simulink model "IEEE68"  (R2024b)
settings: Solver=FixedStepAuto  StartTime=0  StopTime=20  FixedStep=Ts  RelTol=1e-3
undefined symbols (not defined in the file): ApparatusDiscreDamping, ApparatusPara, ApparatusPowerFlow, ApparatusType, Fbase, OtherInputs, Sbase, Ts, Vbase, Wbase, x_e, Ybase, Zbase
libraries: spsGroundLib x101, SimplusGT x98, spsThreePhaseSeriesRLCBranchLib x83, spsThreePhaseParallelRLCBranchLib x71, spsThreePhaseTransformerTwoWindingsLib x16, spsThreePhaseBreakerLib x3, sps_lib x1
settings Model: Creator=tim  LastModifiedBy=tim

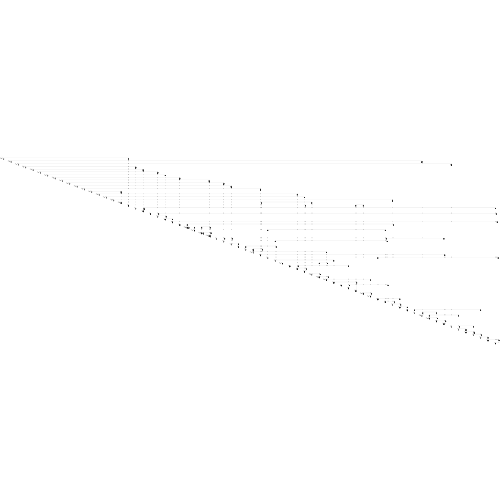
[thumbnail: Simulink's stored preview of the top-level diagram]
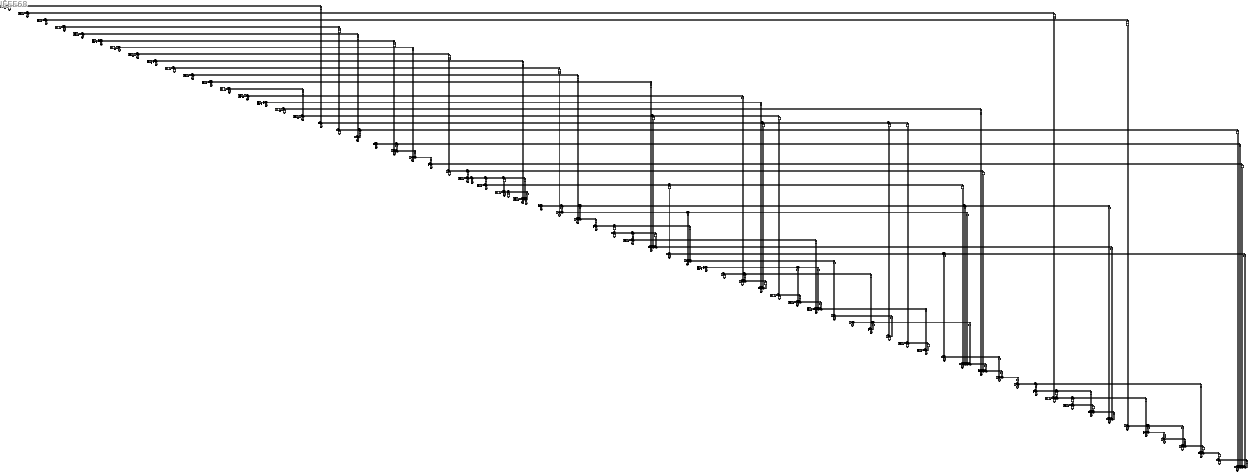
== system IEEE68 ==
  B-GND{1..7,9,11,13,15,17,19,21,23,25,27,29,31,33,36,40,43..44,47,49,51,53,56,60,63,65..66,71,74,76,79,82,84,86,89,91,94,97,99..100,102,104,106,108,111..113,115..116,118,120,122,124,127,130,133,135,137..138,141,143,145,147,149,151} (71 alike) : spsGroundLib/Ground  LConnTagsString=a
  Branch1-1 : spsThreePhaseParallelRLCBranchLib/Three-Phase Parallel RLC Branch  LConnTagsString=A|B|C  RConnTagsString=A|B|C  BranchType=C  Resistance=(Inf)*Zbase  Inductance=(Inf)*Zbase/Wbase  Capacitance=(5e-08)*Ybase/Wbase  Measurements=None
  Branch1-18 : spsThreePhaseSeriesRLCBranchLib/Three-Phase Series RLC Branch  LConnTagsString=A|B|C  RConnTagsString=A|B|C  BranchType=RL  Resistance=(1e-07)*Zbase  Inductance=(0.003)*Zbase/Wbase  Capacitance=1e-6  Measurements=None
  Branch10-10 : spsThreePhaseParallelRLCBranchLib/Three-Phase Parallel RLC Branch  LConnTagsString=A|B|C  RConnTagsString=A|B|C  BranchType=C  Resistance=(Inf)*Zbase  Inductance=(Inf)*Zbase/Wbase  Capacitance=(5e-08)*Ybase/Wbase  Measurements=None
  Branch10-31 : spsThreePhaseSeriesRLCBranchLib/Three-Phase Series RLC Branch  LConnTagsString=A|B|C  RConnTagsString=A|B|C  BranchType=RL  Resistance=(1e-07)*Zbase  Inductance=(0.026)*Zbase/Wbase  Capacitance=1e-6  Measurements=None
  Branch11-11 : spsThreePhaseParallelRLCBranchLib/Three-Phase Parallel RLC Branch  LConnTagsString=A|B|C  RConnTagsString=A|B|C  BranchType=C  Resistance=(Inf)*Zbase  Inductance=(Inf)*Zbase/Wbase  Capacitance=(5e-08)*Ybase/Wbase  Measurements=None
  Branch11-32 : spsThreePhaseSeriesRLCBranchLib/Three-Phase Series RLC Branch  LConnTagsString=A|B|C  RConnTagsString=A|B|C  BranchType=RL  Resistance=(1e-07)*Zbase  Inductance=(0.013)*Zbase/Wbase  Capacitance=1e-6  Measurements=None
  Branch12-12 : spsThreePhaseParallelRLCBranchLib/Three-Phase Parallel RLC Branch  LConnTagsString=A|B|C  RConnTagsString=A|B|C  BranchType=C  Resistance=(Inf)*Zbase  Inductance=(Inf)*Zbase/Wbase  Capacitance=(5e-08)*Ybase/Wbase  Measurements=None
  Branch12-36 : spsThreePhaseSeriesRLCBranchLib/Three-Phase Series RLC Branch  LConnTagsString=A|B|C  RConnTagsString=A|B|C  BranchType=RL  Resistance=(1e-07)*Zbase  Inductance=(0.0075)*Zbase/Wbase  Capacitance=1e-6  Measurements=None
  Branch13-13 : spsThreePhaseParallelRLCBranchLib/Three-Phase Parallel RLC Branch  LConnTagsString=A|B|C  RConnTagsString=A|B|C  BranchType=C  Resistance=(Inf)*Zbase  Inductance=(Inf)*Zbase/Wbase  Capacitance=(5e-08)*Ybase/Wbase  Measurements=None
  Branch13-17 : spsThreePhaseSeriesRLCBranchLib/Three-Phase Series RLC Branch  LConnTagsString=A|B|C  RConnTagsString=A|B|C  BranchType=RL  Resistance=(1e-07)*Zbase  Inductance=(0.0033)*Zbase/Wbase  Capacitance=1e-6  Measurements=None
  Branch14-14 : spsThreePhaseParallelRLCBranchLib/Three-Phase Parallel RLC Branch  LConnTagsString=A|B|C  RConnTagsString=A|B|C  BranchType=C  Resistance=(Inf)*Zbase  Inductance=(Inf)*Zbase/Wbase  Capacitance=(5e-08)*Ybase/Wbase  Measurements=None
  Branch14-41 : spsThreePhaseSeriesRLCBranchLib/Three-Phase Series RLC Branch  LConnTagsString=A|B|C  RConnTagsString=A|B|C  BranchType=RL  Resistance=(1e-07)*Zbase  Inductance=(0.0015)*Zbase/Wbase  Capacitance=1e-6  Measurements=None
  Branch15-15 : spsThreePhaseParallelRLCBranchLib/Three-Phase Parallel RLC Branch  LConnTagsString=A|B|C  RConnTagsString=A|B|C  BranchType=C  Resistance=(Inf)*Zbase  Inductance=(Inf)*Zbase/Wbase  Capacitance=(5e-08)*Ybase/Wbase  Measurements=None
  Branch15-42 : spsThreePhaseSeriesRLCBranchLib/Three-Phase Series RLC Branch  LConnTagsString=A|B|C  RConnTagsString=A|B|C  BranchType=RL  Resistance=(1e-07)*Zbase  Inductance=(0.0015)*Zbase/Wbase  Capacitance=1e-6  Measurements=None
  Branch16-16 : spsThreePhaseParallelRLCBranchLib/Three-Phase Parallel RLC Branch  LConnTagsString=A|B|C  RConnTagsString=A|B|C  BranchType=C  Resistance=(Inf)*Zbase  Inductance=(Inf)*Zbase/Wbase  Capacitance=(5e-08)*Ybase/Wbase  Measurements=None
  Branch16-54 : spsThreePhaseSeriesRLCBranchLib/Three-Phase Series RLC Branch  LConnTagsString=A|B|C  RConnTagsString=A|B|C  BranchType=RL  Resistance=(1e-07)*Zbase  Inductance=(0.0181)*Zbase/Wbase  Capacitance=1e-6  Measurements=None
  Branch17-17 : spsThreePhaseParallelRLCBranchLib/Three-Phase Parallel RLC Branch  LConnTagsString=A|B|C  RConnTagsString=A|B|C  BranchType=RLC  Resistance=(0.014484)*Zbase  Inductance=(0.28969)*Zbase/Wbase  Capacitance=(0.16)*Ybase/Wbase  Measurements=None
  Branch17-36 : spsThreePhaseSeriesRLCBranchLib/Three-Phase Series RLC Branch  LConnTagsString=A|B|C  RConnTagsString=A|B|C  BranchType=RL  Resistance=(0.0005)*Zbase  Inductance=(0.0045)*Zbase/Wbase  Capacitance=1e-6  Measurements=None
  Branch17-43 : spsThreePhaseSeriesRLCBranchLib/Three-Phase Series RLC Branch  LConnTagsString=A|B|C  RConnTagsString=A|B|C  BranchType=RL  Resistance=(0.0005)*Zbase  Inductance=(0.0276)*Zbase/Wbase  Capacitance=1e-6  Measurements=None
  Branch18-18 : spsThreePhaseParallelRLCBranchLib/Three-Phase Parallel RLC Branch  LConnTagsString=A|B|C  RConnTagsString=A|B|C  BranchType=RLC  Resistance=(0.040678)*Zbase  Inductance=(0.81687)*Zbase/Wbase  Capacitance=(2.735)*Ybase/Wbase  Measurements=None
  Branch18-42 : spsThreePhaseSeriesRLCBranchLib/Three-Phase Series RLC Branch  LConnTagsString=A|B|C  RConnTagsString=A|B|C  BranchType=RL  Resistance=(0.004)*Zbase  Inductance=(0.06)*Zbase/Wbase  Capacitance=1e-6  Measurements=None
  Branch18-49 : spsThreePhaseSeriesRLCBranchLib/Three-Phase Series RLC Branch  LConnTagsString=A|B|C  RConnTagsString=A|B|C  BranchType=RL  Resistance=(0.0076)*Zbase  Inductance=(0.1141)*Zbase/Wbase  Capacitance=1e-6  Measurements=None
  Branch18-50 : spsThreePhaseSeriesRLCBranchLib/Three-Phase Series RLC Branch  LConnTagsString=A|B|C  RConnTagsString=A|B|C  BranchType=RL  Resistance=(0.0012)*Zbase  Inductance=(0.0288)*Zbase/Wbase  Capacitance=1e-6  Measurements=None
  Branch19-19 : spsThreePhaseParallelRLCBranchLib/Three-Phase Parallel RLC Branch  LConnTagsString=A|B|C  RConnTagsString=A|B|C  BranchType=C  Resistance=(Inf)*Zbase  Inductance=(Inf)*Zbase/Wbase  Capacitance=(0.152)*Ybase/Wbase  Measurements=None
  Branch19-20 : spsThreePhaseSeriesRLCBranchLib/Three-Phase Series RLC Branch  LConnTagsString=A|B|C  RConnTagsString=A|B|C  BranchType=RL  Resistance=(0.00078652)*Zbase  Inductance=(0.015506)*Zbase/Wbase  Capacitance=1e-6  Measurements=None
  Branch19-68 : spsThreePhaseSeriesRLCBranchLib/Three-Phase Series RLC Branch  LConnTagsString=A|B|C  RConnTagsString=A|B|C  BranchType=RL  Resistance=(0.0016)*Zbase  Inductance=(0.0195)*Zbase/Wbase  Capacitance=1e-6  Measurements=None
  Branch2-2 : spsThreePhaseParallelRLCBranchLib/Three-Phase Parallel RLC Branch  LConnTagsString=A|B|C  RConnTagsString=A|B|C  BranchType=C  Resistance=(Inf)*Zbase  Inductance=(Inf)*Zbase/Wbase  Capacitance=(5e-08)*Ybase/Wbase  Measurements=None
  Branch2-58 : spsThreePhaseSeriesRLCBranchLib/Three-Phase Series RLC Branch  LConnTagsString=A|B|C  RConnTagsString=A|B|C  BranchType=RL  Resistance=(1e-07)*Zbase  Inductance=(0.025)*Zbase/Wbase  Capacitance=1e-6  Measurements=None
  Branch20-20 : spsThreePhaseParallelRLCBranchLib/Three-Phase Parallel RLC Branch  LConnTagsString=A|B|C  RConnTagsString=A|B|C  BranchType=RLC  Resistance=(0.14143)*Zbase  Inductance=(0.9337)*Zbase/Wbase  Capacitance=(1e-07)*Ybase/Wbase  Measurements=None
  Branch21-21 : spsThreePhaseParallelRLCBranchLib/Three-Phase Parallel RLC Branch  LConnTagsString=A|B|C  RConnTagsString=A|B|C  BranchType=RLC  Resistance=(0.33667)*Zbase  Inductance=(0.80214)*Zbase/Wbase  Capacitance=(0.25565)*Ybase/Wbase  Measurements=None
  Branch21-22 : spsThreePhaseSeriesRLCBranchLib/Three-Phase Series RLC Branch  LConnTagsString=A|B|C  RConnTagsString=A|B|C  BranchType=RL  Resistance=(0.0008)*Zbase  Inductance=(0.014)*Zbase/Wbase  Capacitance=1e-6  Measurements=None
  Branch21-68 : spsThreePhaseSeriesRLCBranchLib/Three-Phase Series RLC Branch  LConnTagsString=A|B|C  RConnTagsString=A|B|C  BranchType=RL  Resistance=(0.0008)*Zbase  Inductance=(0.0135)*Zbase/Wbase  Capacitance=1e-6  Measurements=None
  Branch22-22 : spsThreePhaseParallelRLCBranchLib/Three-Phase Parallel RLC Branch  LConnTagsString=A|B|C  RConnTagsString=A|B|C  BranchType=C  Resistance=(Inf)*Zbase  Inductance=(Inf)*Zbase/Wbase  Capacitance=(0.22055)*Ybase/Wbase  Measurements=None
  Branch22-23 : spsThreePhaseSeriesRLCBranchLib/Three-Phase Series RLC Branch  LConnTagsString=A|B|C  RConnTagsString=A|B|C  BranchType=RL  Resistance=(0.0006)*Zbase  Inductance=(0.0096)*Zbase/Wbase  Capacitance=1e-6  Measurements=None
  Branch23-23 : spsThreePhaseParallelRLCBranchLib/Three-Phase Parallel RLC Branch  LConnTagsString=A|B|C  RConnTagsString=A|B|C  BranchType=RLC  Resistance=(0.40019)*Zbase  Inductance=(1.1676)*Zbase/Wbase  Capacitance=(0.2728)*Ybase/Wbase  Measurements=None
  Branch23-24 : spsThreePhaseSeriesRLCBranchLib/Three-Phase Series RLC Branch  LConnTagsString=A|B|C  RConnTagsString=A|B|C  BranchType=RL  Resistance=(0.0022)*Zbase  Inductance=(0.035)*Zbase/Wbase  Capacitance=1e-6  Measurements=None
  Branch24-24 : spsThreePhaseParallelRLCBranchLib/Three-Phase Parallel RLC Branch  LConnTagsString=A|B|C  RConnTagsString=A|B|C  BranchType=RC  Resistance=(0.29761)*Zbase  Inductance=(Inf)*Zbase/Wbase  Capacitance=(1.2149)*Ybase/Wbase  Measurements=None
  Branch24-68 : spsThreePhaseSeriesRLCBranchLib/Three-Phase Series RLC Branch  LConnTagsString=A|B|C  RConnTagsString=A|B|C  BranchType=RL  Resistance=(0.0003)*Zbase  Inductance=(0.0059)*Zbase/Wbase  Capacitance=1e-6  Measurements=None
  Branch25-25 : spsThreePhaseParallelRLCBranchLib/Three-Phase Parallel RLC Branch  LConnTagsString=A|B|C  RConnTagsString=A|B|C  BranchType=RLC  Resistance=(0.44563)*Zbase  Inductance=(2.1238)*Zbase/Wbase  Capacitance=(0.3385)*Ybase/Wbase  Measurements=None
  Branch25-26 : spsThreePhaseSeriesRLCBranchLib/Three-Phase Series RLC Branch  LConnTagsString=A|B|C  RConnTagsString=A|B|C  BranchType=RL  Resistance=(0.0032)*Zbase  Inductance=(0.0323)*Zbase/Wbase  Capacitance=1e-6  Measurements=None
  Branch25-54 : spsThreePhaseSeriesRLCBranchLib/Three-Phase Series RLC Branch  LConnTagsString=A|B|C  RConnTagsString=A|B|C  BranchType=RL  Resistance=(0.007)*Zbase  Inductance=(0.0086)*Zbase/Wbase  Capacitance=1e-6  Measurements=None
  Branch26-1 : spsThreePhaseParallelRLCBranchLib/Three-Phase Parallel RLC Branch  LConnTagsString=A|B|C  RConnTagsString=A|B|C  BranchType=R  Resistance=(0.71464)*Zbase*4  Inductance=(5.8432)*Zbase/Wbase  Capacitance=(1.2899)*Ybase/Wbase  Measurements=None
  Branch26-2 : spsThreePhaseParallelRLCBranchLib/Three-Phase Parallel RLC Branch  LConnTagsString=A|B|C  RConnTagsString=A|B|C  BranchType=R  Resistance=(0.49017)*Zbase*4  Inductance=(5.8432)*Zbase/Wbase  Capacitance=(1.2899)*Ybase/Wbase  Measurements=None
  Branch26-26 : spsThreePhaseParallelRLCBranchLib/Three-Phase Parallel RLC Branch  LConnTagsString=A|B|C  RConnTagsString=A|B|C  BranchType=RLC  Resistance=(0.71464)*Zbase  Inductance=(5.8432)*Zbase/Wbase  Capacitance=(1.2899)*Ybase/Wbase  Measurements=None
  Branch26-27 : spsThreePhaseSeriesRLCBranchLib/Three-Phase Series RLC Branch  LConnTagsString=A|B|C  RConnTagsString=A|B|C  BranchType=RL  Resistance=(0.0014)*Zbase  Inductance=(0.0147)*Zbase/Wbase  Capacitance=1e-6  Measurements=None
  Branch26-28 : spsThreePhaseSeriesRLCBranchLib/Three-Phase Series RLC Branch  LConnTagsString=A|B|C  RConnTagsString=A|B|C  BranchType=RL  Resistance=(0.0043)*Zbase  Inductance=(0.0474)*Zbase/Wbase  Capacitance=1e-6  Measurements=None
  Branch26-29 : spsThreePhaseSeriesRLCBranchLib/Three-Phase Series RLC Branch  LConnTagsString=A|B|C  RConnTagsString=A|B|C  BranchType=RL  Resistance=(0.0057)*Zbase  Inductance=(0.0625)*Zbase/Wbase  Capacitance=1e-6  Measurements=None
  Branch26-3 : spsThreePhaseParallelRLCBranchLib/Three-Phase Parallel RLC Branch  LConnTagsString=A|B|C  RConnTagsString=A|B|C  BranchType=R  Resistance=(0.35501)*Zbase*4  Inductance=(5.8432)*Zbase/Wbase  Capacitance=(1.2899)*Ybase/Wbase  Measurements=None
  Branch27-27 : spsThreePhaseParallelRLCBranchLib/Three-Phase Parallel RLC Branch  LConnTagsString=A|B|C  RConnTagsString=A|B|C  BranchType=RLC  Resistance=(0.3379)*Zbase  Inductance=(1.2493)*Zbase/Wbase  Capacitance=(0.4856)*Ybase/Wbase  Measurements=None
  Branch27-37 : spsThreePhaseSeriesRLCBranchLib/Three-Phase Series RLC Branch  LConnTagsString=A|B|C  RConnTagsString=A|B|C  BranchType=RL  Resistance=(0.0013)*Zbase  Inductance=(0.0173)*Zbase/Wbase  Capacitance=1e-6  Measurements=None
  Branch27-53 : spsThreePhaseSeriesRLCBranchLib/Three-Phase Series RLC Branch  LConnTagsString=A|B|C  RConnTagsString=A|B|C  BranchType=RL  Resistance=(0.032)*Zbase  Inductance=(0.32)*Zbase/Wbase  Capacitance=1e-6  Measurements=None
  Branch28-28 : spsThreePhaseParallelRLCBranchLib/Three-Phase Parallel RLC Branch  LConnTagsString=A|B|C  RConnTagsString=A|B|C  BranchType=RLC  Resistance=(0.49017)*Zbase  Inductance=(3.6062)*Zbase/Wbase  Capacitance=(0.5146)*Ybase/Wbase  Measurements=None
  Branch28-29 : spsThreePhaseSeriesRLCBranchLib/Three-Phase Series RLC Branch  LConnTagsString=A|B|C  RConnTagsString=A|B|C  BranchType=RL  Resistance=(0.0014)*Zbase  Inductance=(0.0151)*Zbase/Wbase  Capacitance=1e-6  Measurements=None
  Branch29-29 : spsThreePhaseParallelRLCBranchLib/Three-Phase Parallel RLC Branch  LConnTagsString=A|B|C  RConnTagsString=A|B|C  BranchType=RLC  Resistance=(0.35501)*Zbase  Inductance=(3.7342)*Zbase/Wbase  Capacitance=(0.639)*Ybase/Wbase  Measurements=None
  Branch3-3 : spsThreePhaseParallelRLCBranchLib/Three-Phase Parallel RLC Branch  LConnTagsString=A|B|C  RConnTagsString=A|B|C  BranchType=C  Resistance=(Inf)*Zbase  Inductance=(Inf)*Zbase/Wbase  Capacitance=(5e-08)*Ybase/Wbase  Measurements=None
  Branch3-62 : spsThreePhaseSeriesRLCBranchLib/Three-Phase Series RLC Branch  LConnTagsString=A|B|C  RConnTagsString=A|B|C  BranchType=RL  Resistance=(1e-07)*Zbase  Inductance=(0.02)*Zbase/Wbase  Capacitance=1e-6  Measurements=None
  Branch30-30 : spsThreePhaseParallelRLCBranchLib/Three-Phase Parallel RLC Branch  LConnTagsString=A|B|C  RConnTagsString=A|B|C  BranchType=C  Resistance=(Inf)*Zbase  Inductance=(Inf)*Zbase/Wbase  Capacitance=(0.9405)*Ybase/Wbase  Measurements=None
  Branch30-31 : spsThreePhaseSeriesRLCBranchLib/Three-Phase Series RLC Branch  LConnTagsString=A|B|C  RConnTagsString=A|B|C  BranchType=RL  Resistance=(0.0013)*Zbase  Inductance=(0.0187)*Zbase/Wbase  Capacitance=1e-6  Measurements=None
  Branch30-32 : spsThreePhaseSeriesRLCBranchLib/Three-Phase Series RLC Branch  LConnTagsString=A|B|C  RConnTagsString=A|B|C  BranchType=RL  Resistance=(0.0024)*Zbase  Inductance=(0.0288)*Zbase/Wbase  Capacitance=1e-6  Measurements=None
  Branch30-53 : spsThreePhaseSeriesRLCBranchLib/Three-Phase Series RLC Branch  LConnTagsString=A|B|C  RConnTagsString=A|B|C  BranchType=RL  Resistance=(0.0008)*Zbase  Inductance=(0.0074)*Zbase/Wbase  Capacitance=1e-6  Measurements=None
  Branch30-61 : spsThreePhaseSeriesRLCBranchLib/Three-Phase Series RLC Branch  LConnTagsString=A|B|C  RConnTagsString=A|B|C  BranchType=RL  Resistance=(0.00095)*Zbase  Inductance=(0.00915)*Zbase/Wbase  Capacitance=1e-6  Measurements=None
  Branch31-31 : spsThreePhaseParallelRLCBranchLib/Three-Phase Parallel RLC Branch  LConnTagsString=A|B|C  RConnTagsString=A|B|C  BranchType=C  Resistance=(Inf)*Zbase  Inductance=(Inf)*Zbase/Wbase  Capacitance=(0.415)*Ybase/Wbase  Measurements=None
  Branch31-38 : spsThreePhaseSeriesRLCBranchLib/Three-Phase Series RLC Branch  LConnTagsString=A|B|C  RConnTagsString=A|B|C  BranchType=RL  Resistance=(0.0011)*Zbase  Inductance=(0.0147)*Zbase/Wbase  Capacitance=1e-6  Measurements=None
  Branch31-53 : spsThreePhaseSeriesRLCBranchLib/Three-Phase Series RLC Branch  LConnTagsString=A|B|C  RConnTagsString=A|B|C  BranchType=RL  Resistance=(0.0016)*Zbase  Inductance=(0.0163)*Zbase/Wbase  Capacitance=1e-6  Measurements=None
  Branch32-32 : spsThreePhaseParallelRLCBranchLib/Three-Phase Parallel RLC Branch  LConnTagsString=A|B|C  RConnTagsString=A|B|C  BranchType=C  Resistance=(Inf)*Zbase  Inductance=(Inf)*Zbase/Wbase  Capacitance=(0.328)*Ybase/Wbase  Measurements=None
  Branch32-33 : spsThreePhaseSeriesRLCBranchLib/Three-Phase Series RLC Branch  LConnTagsString=A|B|C  RConnTagsString=A|B|C  BranchType=RL  Resistance=(0.0008)*Zbase  Inductance=(0.0099)*Zbase/Wbase  Capacitance=1e-6  Measurements=None
  Branch33-33 : spsThreePhaseParallelRLCBranchLib/Three-Phase Parallel RLC Branch  LConnTagsString=A|B|C  RConnTagsString=A|B|C  BranchType=RC  Resistance=(0.82543)*Zbase  Inductance=(Inf)*Zbase/Wbase  Capacitance=(0.5315)*Ybase/Wbase  Measurements=None
  Branch33-34 : spsThreePhaseSeriesRLCBranchLib/Three-Phase Series RLC Branch  LConnTagsString=A|B|C  RConnTagsString=A|B|C  BranchType=RL  Resistance=(0.0011)*Zbase  Inductance=(0.0157)*Zbase/Wbase  Capacitance=1e-6  Measurements=None
  Branch33-38 : spsThreePhaseSeriesRLCBranchLib/Three-Phase Series RLC Branch  LConnTagsString=A|B|C  RConnTagsString=A|B|C  BranchType=RL  Resistance=(0.0036)*Zbase  Inductance=(0.0444)*Zbase/Wbase  Capacitance=1e-6  Measurements=None
  Branch34-34 : spsThreePhaseParallelRLCBranchLib/Three-Phase Parallel RLC Branch  LConnTagsString=A|B|C  RConnTagsString=A|B|C  BranchType=C  Resistance=(Inf)*Zbase  Inductance=(Inf)*Zbase/Wbase  Capacitance=(0.826)*Ybase/Wbase  Measurements=None
  Branch34-35 : spsThreePhaseSeriesRLCBranchLib/Three-Phase Series RLC Branch  LConnTagsString=A|B|C  RConnTagsString=A|B|C  BranchType=RL  Resistance=(0.0001)*Zbase  Inductance=(0.0074)*Zbase/Wbase  Capacitance=1e-6  Measurements=None
  Branch34-36 : spsThreePhaseSeriesRLCBranchLib/Three-Phase Series RLC Branch  LConnTagsString=A|B|C  RConnTagsString=A|B|C  BranchType=RL  Resistance=(0.0033)*Zbase  Inductance=(0.0111)*Zbase/Wbase  Capacitance=1e-6  Measurements=None
  Branch35-35 : spsThreePhaseParallelRLCBranchLib/Three-Phase Parallel RLC Branch  LConnTagsString=A|B|C  RConnTagsString=A|B|C  BranchType=C  Resistance=(Inf)*Zbase  Inductance=(Inf)*Zbase/Wbase  Capacitance=(0.695)*Ybase/Wbase  Measurements=None
  Branch35-45 : spsThreePhaseSeriesRLCBranchLib/Three-Phase Series RLC Branch  LConnTagsString=A|B|C  RConnTagsString=A|B|C  BranchType=RL  Resistance=(0.0007)*Zbase  Inductance=(0.0175)*Zbase/Wbase  Capacitance=1e-6  Measurements=None
  Branch36-36 : spsThreePhaseParallelRLCBranchLib/Three-Phase Parallel RLC Branch  LConnTagsString=A|B|C  RConnTagsString=A|B|C  BranchType=RC  Resistance=(0.84882)*Zbase  Inductance=(Inf)*Zbase/Wbase  Capacitance=(1.4498)*Ybase/Wbase  Measurements=None
  Branch36-61 : spsThreePhaseSeriesRLCBranchLib/Three-Phase Series RLC Branch  LConnTagsString=A|B|C  RConnTagsString=A|B|C  BranchType=RL  Resistance=(0.0011)*Zbase  Inductance=(0.0098)*Zbase/Wbase  Capacitance=1e-6  Measurements=None
  Branch37-37 : spsThreePhaseParallelRLCBranchLib/Three-Phase Parallel RLC Branch  LConnTagsString=A|B|C  RConnTagsString=A|B|C  BranchType=C  Resistance=(Inf)*Zbase  Inductance=(Inf)*Zbase/Wbase  Capacitance=(0.29385)*Ybase/Wbase  Measurements=None
  Branch37-52 : spsThreePhaseSeriesRLCBranchLib/Three-Phase Series RLC Branch  LConnTagsString=A|B|C  RConnTagsString=A|B|C  BranchType=RL  Resistance=(0.0007)*Zbase  Inductance=(0.0082)*Zbase/Wbase  Capacitance=1e-6  Measurements=None
  Branch37-68 : spsThreePhaseSeriesRLCBranchLib/Three-Phase Series RLC Branch  LConnTagsString=A|B|C  RConnTagsString=A|B|C  BranchType=RL  Resistance=(0.0007)*Zbase  Inductance=(0.0089)*Zbase/Wbase  Capacitance=1e-6  Measurements=None
  Branch38-38 : spsThreePhaseParallelRLCBranchLib/Three-Phase Parallel RLC Branch  LConnTagsString=A|B|C  RConnTagsString=A|B|C  BranchType=C  Resistance=(Inf)*Zbase  Inductance=(Inf)*Zbase/Wbase  Capacitance=(0.685)*Ybase/Wbase  Measurements=None
  Branch38-46 : spsThreePhaseSeriesRLCBranchLib/Three-Phase Series RLC Branch  LConnTagsString=A|B|C  RConnTagsString=A|B|C  BranchType=RL  Resistance=(0.0022)*Zbase  Inductance=(0.0284)*Zbase/Wbase  Capacitance=1e-6  Measurements=None
  Branch39-39 : spsThreePhaseParallelRLCBranchLib/Three-Phase Parallel RLC Branch  LConnTagsString=A|B|C  RConnTagsString=A|B|C  BranchType=RLC  Resistance=(0.38369)*Zbase  Inductance=(8.1305)*Zbase/Wbase  Capacitance=(1e-07)*Ybase/Wbase  Measurements=None
  Branch39-44 : spsThreePhaseSeriesRLCBranchLib/Three-Phase Series RLC Branch  LConnTagsString=A|B|C  RConnTagsString=A|B|C  BranchType=RL  Resistance=(1e-07)*Zbase  Inductance=(0.0411)*Zbase/Wbase  Capacitance=1e-6  Measurements=None
  Branch39-45 : spsThreePhaseSeriesRLCBranchLib/Three-Phase Series RLC Branch  LConnTagsString=A|B|C  RConnTagsString=A|B|C  BranchType=RL  Resistance=(1e-07)*Zbase  Inductance=(0.0839)*Zbase/Wbase  Capacitance=1e-6  Measurements=None
  Branch4-19 : spsThreePhaseSeriesRLCBranchLib/Three-Phase Series RLC Branch  LConnTagsString=A|B|C  RConnTagsString=A|B|C  BranchType=RL  Resistance=(0.0007)*Zbase  Inductance=(0.0142)*Zbase/Wbase  Capacitance=1e-6  Measurements=None
  Branch4-4 : spsThreePhaseParallelRLCBranchLib/Three-Phase Parallel RLC Branch  LConnTagsString=A|B|C  RConnTagsString=A|B|C  BranchType=C  Resistance=(Inf)*Zbase  Inductance=(Inf)*Zbase/Wbase  Capacitance=(5e-08)*Ybase/Wbase  Measurements=None
  Branch40-40 : spsThreePhaseParallelRLCBranchLib/Three-Phase Parallel RLC Branch  LConnTagsString=A|B|C  RConnTagsString=A|B|C  BranchType=RLC  Resistance=(1.513)*Zbase  Inductance=(4.22)*Zbase/Wbase  Capacitance=(2.215)*Ybase/Wbase  Measurements=None
  Branch40-41 : spsThreePhaseSeriesRLCBranchLib/Three-Phase Series RLC Branch  LConnTagsString=A|B|C  RConnTagsString=A|B|C  BranchType=RL  Resistance=(0.006)*Zbase  Inductance=(0.084)*Zbase/Wbase  Capacitance=1e-6  Measurements=None
  Branch40-48 : spsThreePhaseSeriesRLCBranchLib/Three-Phase Series RLC Branch  LConnTagsString=A|B|C  RConnTagsString=A|B|C  BranchType=RL  Resistance=(0.002)*Zbase  Inductance=(0.022)*Zbase/Wbase  Capacitance=1e-6  Measurements=None
  Branch41-41 : spsThreePhaseParallelRLCBranchLib/Three-Phase Parallel RLC Branch  LConnTagsString=A|B|C  RConnTagsString=A|B|C  BranchType=RLC  Resistance=(0.099656)*Zbase  Inductance=(0.39863)*Zbase/Wbase  Capacitance=(2.7)*Ybase/Wbase  Measurements=None
  Branch41-42 : spsThreePhaseSeriesRLCBranchLib/Three-Phase Series RLC Branch  LConnTagsString=A|B|C  RConnTagsString=A|B|C  BranchType=RL  Resistance=(0.004)*Zbase  Inductance=(0.06)*Zbase/Wbase  Capacitance=1e-6  Measurements=None
  Branch42-42 : spsThreePhaseParallelRLCBranchLib/Three-Phase Parallel RLC Branch  LConnTagsString=A|B|C  RConnTagsString=A|B|C  BranchType=RLC  Resistance=(0.086822)*Zbase  Inductance=(0.39938)*Zbase/Wbase  Capacitance=(2.25)*Ybase/Wbase  Measurements=None
  Branch43-43 : spsThreePhaseParallelRLCBranchLib/Three-Phase Parallel RLC Branch  LConnTagsString=A|B|C  RConnTagsString=A|B|C  BranchType=C  Resistance=(Inf)*Zbase  Inductance=(Inf)*Zbase/Wbase  Capacitance=(1e-07)*Ybase/Wbase  Measurements=None
  Branch43-44 : spsThreePhaseSeriesRLCBranchLib/Three-Phase Series RLC Branch  LConnTagsString=A|B|C  RConnTagsString=A|B|C  BranchType=RL  Resistance=(0.0001)*Zbase  Inductance=(0.0011)*Zbase/Wbase  Capacitance=1e-6  Measurements=None
  Branch44-44 : spsThreePhaseParallelRLCBranchLib/Three-Phase Parallel RLC Branch  LConnTagsString=A|B|C  RConnTagsString=A|B|C  BranchType=RLC  Resistance=(0.35162)*Zbase  Inductance=(19.4374)*Zbase/Wbase  Capacitance=(1.5e-07)*Ybase/Wbase  Measurements=None
  Branch44-45 : spsThreePhaseSeriesRLCBranchLib/Three-Phase Series RLC Branch  LConnTagsString=A|B|C  RConnTagsString=A|B|C  BranchType=RL  Resistance=(0.0025)*Zbase  Inductance=(0.073)*Zbase/Wbase  Capacitance=1e-6  Measurements=None
  Branch45-45 : spsThreePhaseParallelRLCBranchLib/Three-Phase Parallel RLC Branch  LConnTagsString=A|B|C  RConnTagsString=A|B|C  BranchType=RLC  Resistance=(0.52088)*Zbase  Inductance=(5.1592)*Zbase/Wbase  Capacitance=(1.055)*Ybase/Wbase  Measurements=None
  Branch45-51 : spsThreePhaseSeriesRLCBranchLib/Three-Phase Series RLC Branch  LConnTagsString=A|B|C  RConnTagsString=A|B|C  BranchType=RL  Resistance=(0.0004)*Zbase  Inductance=(0.0105)*Zbase/Wbase  Capacitance=1e-6  Measurements=None
  Branch46-46 : spsThreePhaseParallelRLCBranchLib/Three-Phase Parallel RLC Branch  LConnTagsString=A|B|C  RConnTagsString=A|B|C  BranchType=RLC  Resistance=(0.60968)*Zbase  Inductance=(3.2238)*Zbase/Wbase  Capacitance=(0.35)*Ybase/Wbase  Measurements=None
  Branch46-49 : spsThreePhaseSeriesRLCBranchLib/Three-Phase Series RLC Branch  LConnTagsString=A|B|C  RConnTagsString=A|B|C  BranchType=RL  Resistance=(0.0018)*Zbase  Inductance=(0.0274)*Zbase/Wbase  Capacitance=1e-6  Measurements=None
  Branch47-47 : spsThreePhaseParallelRLCBranchLib/Three-Phase Parallel RLC Branch  LConnTagsString=A|B|C  RConnTagsString=A|B|C  BranchType=RLC  Resistance=(0.47479)*Zbase  Inductance=(2.9591)*Zbase/Wbase  Capacitance=(1.055)*Ybase/Wbase  Measurements=None
  Branch47-48 : spsThreePhaseSeriesRLCBranchLib/Three-Phase Series RLC Branch  LConnTagsString=A|B|C  RConnTagsString=A|B|C  BranchType=RL  Resistance=(0.00125)*Zbase  Inductance=(0.0134)*Zbase/Wbase  Capacitance=1e-6  Measurements=None
  Branch47-53 : spsThreePhaseSeriesRLCBranchLib/Three-Phase Series RLC Branch  LConnTagsString=A|B|C  RConnTagsString=A|B|C  BranchType=RL  Resistance=(0.0013)*Zbase  Inductance=(0.0188)*Zbase/Wbase  Capacitance=1e-6  Measurements=None
  Branch48-48 : spsThreePhaseParallelRLCBranchLib/Three-Phase Parallel RLC Branch  LConnTagsString=A|B|C  RConnTagsString=A|B|C  BranchType=RLC  Resistance=(0.40748)*Zbase  Inductance=(44.6749)*Zbase/Wbase  Capacitance=(1.04)*Ybase/Wbase  Measurements=None
  Branch49-49 : spsThreePhaseParallelRLCBranchLib/Three-Phase Parallel RLC Branch  LConnTagsString=A|B|C  RConnTagsString=A|B|C  BranchType=RLC  Resistance=(0.55479)*Zbase  Inductance=(3.1374)*Zbase/Wbase  Capacitance=(0.715)*Ybase/Wbase  Measurements=None
  Branch5-20 : spsThreePhaseSeriesRLCBranchLib/Three-Phase Series RLC Branch  LConnTagsString=A|B|C  RConnTagsString=A|B|C  BranchType=RL  Resistance=(0.0009)*Zbase  Inductance=(0.018)*Zbase/Wbase  Capacitance=1e-6  Measurements=None
  Branch5-5 : spsThreePhaseParallelRLCBranchLib/Three-Phase Parallel RLC Branch  LConnTagsString=A|B|C  RConnTagsString=A|B|C  BranchType=C  Resistance=(Inf)*Zbase  Inductance=(Inf)*Zbase/Wbase  Capacitance=(5e-08)*Ybase/Wbase  Measurements=None
  Branch50-50 : spsThreePhaseParallelRLCBranchLib/Three-Phase Parallel RLC Branch  LConnTagsString=A|B|C  RConnTagsString=A|B|C  BranchType=RC  Resistance=(1.1414)*Zbase  Inductance=(Inf)*Zbase/Wbase  Capacitance=(3.1279)*Ybase/Wbase  Measurements=None
  Branch50-51 : spsThreePhaseSeriesRLCBranchLib/Three-Phase Series RLC Branch  LConnTagsString=A|B|C  RConnTagsString=A|B|C  BranchType=RL  Resistance=(0.0009)*Zbase  Inductance=(0.0221)*Zbase/Wbase  Capacitance=1e-6  Measurements=None
  Branch51-51 : spsThreePhaseParallelRLCBranchLib/Three-Phase Parallel RLC Branch  LConnTagsString=A|B|C  RConnTagsString=A|B|C  BranchType=RC  Resistance=(0.33422)*Zbase  Inductance=(Inf)*Zbase/Wbase  Capacitance=(2.2532)*Ybase/Wbase  Measurements=None
  Branch52-52 : spsThreePhaseParallelRLCBranchLib/Three-Phase Parallel RLC Branch  LConnTagsString=A|B|C  RConnTagsString=A|B|C  BranchType=RLC  Resistance=(0.57615)*Zbase  Inductance=(3.0344)*Zbase/Wbase  Capacitance=(0.17285)*Ybase/Wbase  Measurements=None
  Branch52-55 : spsThreePhaseSeriesRLCBranchLib/Three-Phase Series RLC Branch  LConnTagsString=A|B|C  RConnTagsString=A|B|C  BranchType=RL  Resistance=(0.0011)*Zbase  Inductance=(0.0133)*Zbase/Wbase  Capacitance=1e-6  Measurements=None
  Branch53-53 : spsThreePhaseParallelRLCBranchLib/Three-Phase Parallel RLC Branch  LConnTagsString=A|B|C  RConnTagsString=A|B|C  BranchType=RLC  Resistance=(0.36501)*Zbase  Inductance=(0.77798)*Zbase/Wbase  Capacitance=(1.5744)*Ybase/Wbase  Measurements=None
  Branch53-54 : spsThreePhaseSeriesRLCBranchLib/Three-Phase Series RLC Branch  LConnTagsString=A|B|C  RConnTagsString=A|B|C  BranchType=RL  Resistance=(0.0035)*Zbase  Inductance=(0.0411)*Zbase/Wbase  Capacitance=1e-6  Measurements=None
  Branch54-54 : spsThreePhaseParallelRLCBranchLib/Three-Phase Parallel RLC Branch  LConnTagsString=A|B|C  RConnTagsString=A|B|C  BranchType=C  Resistance=(Inf)*Zbase  Inductance=(Inf)*Zbase/Wbase  Capacitance=(0.55095)*Ybase/Wbase  Measurements=None
  Branch54-55 : spsThreePhaseSeriesRLCBranchLib/Three-Phase Series RLC Branch  LConnTagsString=A|B|C  RConnTagsString=A|B|C  BranchType=RL  Resistance=(0.0013)*Zbase  Inductance=(0.0151)*Zbase/Wbase  Capacitance=1e-6  Measurements=None
  Branch55-55 : spsThreePhaseParallelRLCBranchLib/Three-Phase Parallel RLC Branch  LConnTagsString=A|B|C  RConnTagsString=A|B|C  BranchType=RLC  Resistance=(0.28275)*Zbase  Inductance=(45.522)*Zbase/Wbase  Capacitance=(0.3462)*Ybase/Wbase  Measurements=None
  Branch55-56 : spsThreePhaseSeriesRLCBranchLib/Three-Phase Series RLC Branch  LConnTagsString=A|B|C  RConnTagsString=A|B|C  BranchType=RL  Resistance=(0.0013)*Zbase  Inductance=(0.0213)*Zbase/Wbase  Capacitance=1e-6  Measurements=None
  Branch56-56 : spsThreePhaseParallelRLCBranchLib/Three-Phase Parallel RLC Branch  LConnTagsString=A|B|C  RConnTagsString=A|B|C  BranchType=RLC  Resistance=(0.42057)*Zbase  Inductance=(1.1429)*Zbase/Wbase  Capacitance=(0.2469)*Ybase/Wbase  Measurements=None
  Branch56-57 : spsThreePhaseSeriesRLCBranchLib/Three-Phase Series RLC Branch  LConnTagsString=A|B|C  RConnTagsString=A|B|C  BranchType=RL  Resistance=(0.0008)*Zbase  Inductance=(0.0128)*Zbase/Wbase  Capacitance=1e-6  Measurements=None
  Branch56-66 : spsThreePhaseSeriesRLCBranchLib/Three-Phase Series RLC Branch  LConnTagsString=A|B|C  RConnTagsString=A|B|C  BranchType=RL  Resistance=(0.0008)*Zbase  Inductance=(0.0129)*Zbase/Wbase  Capacitance=1e-6  Measurements=None
  Branch57-57 : spsThreePhaseParallelRLCBranchLib/Three-Phase Parallel RLC Branch  LConnTagsString=A|B|C  RConnTagsString=A|B|C  BranchType=C  Resistance=(Inf)*Zbase  Inductance=(Inf)*Zbase/Wbase  Capacitance=(0.1626)*Ybase/Wbase  Measurements=None
  Branch57-58 : spsThreePhaseSeriesRLCBranchLib/Three-Phase Series RLC Branch  LConnTagsString=A|B|C  RConnTagsString=A|B|C  BranchType=RL  Resistance=(0.0002)*Zbase  Inductance=(0.0026)*Zbase/Wbase  Capacitance=1e-6  Measurements=None
  Branch57-60 : spsThreePhaseSeriesRLCBranchLib/Three-Phase Series RLC Branch  LConnTagsString=A|B|C  RConnTagsString=A|B|C  BranchType=RL  Resistance=(0.0008)*Zbase  Inductance=(0.0112)*Zbase/Wbase  Capacitance=1e-6  Measurements=None
  Branch58-58 : spsThreePhaseParallelRLCBranchLib/Three-Phase Parallel RLC Branch  LConnTagsString=A|B|C  RConnTagsString=A|B|C  BranchType=C  Resistance=(Inf)*Zbase  Inductance=(Inf)*Zbase/Wbase  Capacitance=(0.14765)*Ybase/Wbase  Measurements=None
  Branch58-59 : spsThreePhaseSeriesRLCBranchLib/Three-Phase Series RLC Branch  LConnTagsString=A|B|C  RConnTagsString=A|B|C  BranchType=RL  Resistance=(0.0006)*Zbase  Inductance=(0.0092)*Zbase/Wbase  Capacitance=1e-6  Measurements=None
  Branch58-63 : spsThreePhaseSeriesRLCBranchLib/Three-Phase Series RLC Branch  LConnTagsString=A|B|C  RConnTagsString=A|B|C  BranchType=RL  Resistance=(0.0007)*Zbase  Inductance=(0.0082)*Zbase/Wbase  Capacitance=1e-6  Measurements=None
  Branch59-59 : spsThreePhaseParallelRLCBranchLib/Three-Phase Parallel RLC Branch  LConnTagsString=A|B|C  RConnTagsString=A|B|C  BranchType=RLC  Resistance=(0.34307)*Zbase  Inductance=(0.9557)*Zbase/Wbase  Capacitance=(0.0955)*Ybase/Wbase  Measurements=None
  Branch59-60 : spsThreePhaseSeriesRLCBranchLib/Three-Phase Series RLC Branch  LConnTagsString=A|B|C  RConnTagsString=A|B|C  BranchType=RL  Resistance=(0.0004)*Zbase  Inductance=(0.0046)*Zbase/Wbase  Capacitance=1e-6  Measurements=None
  Branch6-22 : spsThreePhaseSeriesRLCBranchLib/Three-Phase Series RLC Branch  LConnTagsString=A|B|C  RConnTagsString=A|B|C  BranchType=RL  Resistance=(1e-07)*Zbase  Inductance=(0.0143)*Zbase/Wbase  Capacitance=1e-6  Measurements=None
  Branch6-6 : spsThreePhaseParallelRLCBranchLib/Three-Phase Parallel RLC Branch  LConnTagsString=A|B|C  RConnTagsString=A|B|C  BranchType=C  Resistance=(Inf)*Zbase  Inductance=(Inf)*Zbase/Wbase  Capacitance=(5e-08)*Ybase/Wbase  Measurements=None
  Branch60-60 : spsThreePhaseParallelRLCBranchLib/Three-Phase Parallel RLC Branch  LConnTagsString=A|B|C  RConnTagsString=A|B|C  BranchType=RLC  Resistance=(0.38448)*Zbase  Inductance=(1.1339)*Zbase/Wbase  Capacitance=(0.303)*Ybase/Wbase  Measurements=None
  Branch60-61 : spsThreePhaseSeriesRLCBranchLib/Three-Phase Series RLC Branch  LConnTagsString=A|B|C  RConnTagsString=A|B|C  BranchType=RL  Resistance=(0.0023)*Zbase  Inductance=(0.0363)*Zbase/Wbase  Capacitance=1e-6  Measurements=None
  Branch61-61 : spsThreePhaseParallelRLCBranchLib/Three-Phase Parallel RLC Branch  LConnTagsString=A|B|C  RConnTagsString=A|B|C  BranchType=RLC  Resistance=(0.82011)*Zbase  Inductance=(0.68233)*Zbase/Wbase  Capacitance=(0.8202)*Ybase/Wbase  Measurements=None
  Branch62-62 : spsThreePhaseParallelRLCBranchLib/Three-Phase Parallel RLC Branch  LConnTagsString=A|B|C  RConnTagsString=A|B|C  BranchType=C  Resistance=(Inf)*Zbase  Inductance=(Inf)*Zbase/Wbase  Capacitance=(0.0729)*Ybase/Wbase  Measurements=None
  Branch62-63 : spsThreePhaseSeriesRLCBranchLib/Three-Phase Series RLC Branch  LConnTagsString=A|B|C  RConnTagsString=A|B|C  BranchType=RL  Resistance=(0.0004)*Zbase  Inductance=(0.0043)*Zbase/Wbase  Capacitance=1e-6  Measurements=None
  Branch62-65 : spsThreePhaseSeriesRLCBranchLib/Three-Phase Series RLC Branch  LConnTagsString=A|B|C  RConnTagsString=A|B|C  BranchType=RL  Resistance=(0.0004)*Zbase  Inductance=(0.0043)*Zbase/Wbase  Capacitance=1e-6  Measurements=None
  Branch63-63 : spsThreePhaseParallelRLCBranchLib/Three-Phase Parallel RLC Branch  LConnTagsString=A|B|C  RConnTagsString=A|B|C  BranchType=C  Resistance=(Inf)*Zbase  Inductance=(Inf)*Zbase/Wbase  Capacitance=(0.1059)*Ybase/Wbase  Measurements=None
  Branch63-64 : spsThreePhaseSeriesRLCBranchLib/Three-Phase Series RLC Branch  LConnTagsString=A|B|C  RConnTagsString=A|B|C  BranchType=RL  Resistance=(0.0016)*Zbase  Inductance=(0.0435)*Zbase/Wbase  Capacitance=1e-6  Measurements=None
  Branch64-64 : spsThreePhaseParallelRLCBranchLib/Three-Phase Parallel RLC Branch  LConnTagsString=A|B|C  RConnTagsString=A|B|C  BranchType=RLC  Resistance=(7.7218)*Zbase  Inductance=(0.78973)*Zbase/Wbase  Capacitance=(1e-07)*Ybase/Wbase  Measurements=None
  Branch64-65 : spsThreePhaseSeriesRLCBranchLib/Three-Phase Series RLC Branch  LConnTagsString=A|B|C  RConnTagsString=A|B|C  BranchType=RL  Resistance=(0.0017978)*Zbase  Inductance=(0.048877)*Zbase/Wbase  Capacitance=1e-6  Measurements=None
  Branch65-65 : spsThreePhaseParallelRLCBranchLib/Three-Phase Parallel RLC Branch  LConnTagsString=A|B|C  RConnTagsString=A|B|C  BranchType=C  Resistance=(Inf)*Zbase  Inductance=(Inf)*Zbase/Wbase  Capacitance=(0.1226)*Ybase/Wbase  Measurements=None
  Branch65-66 : spsThreePhaseSeriesRLCBranchLib/Three-Phase Series RLC Branch  LConnTagsString=A|B|C  RConnTagsString=A|B|C  BranchType=RL  Resistance=(0.0009)*Zbase  Inductance=(0.0101)*Zbase/Wbase  Capacitance=1e-6  Measurements=None
  Branch66-66 : spsThreePhaseParallelRLCBranchLib/Three-Phase Parallel RLC Branch  LConnTagsString=A|B|C  RConnTagsString=A|B|C  BranchType=C  Resistance=(Inf)*Zbase  Inductance=(Inf)*Zbase/Wbase  Capacitance=(0.33825)*Ybase/Wbase  Measurements=None
  Branch66-67 : spsThreePhaseSeriesRLCBranchLib/Three-Phase Series RLC Branch  LConnTagsString=A|B|C  RConnTagsString=A|B|C  BranchType=RL  Resistance=(0.0018)*Zbase  Inductance=(0.0217)*Zbase/Wbase  Capacitance=1e-6  Measurements=None
  Branch67-67 : spsThreePhaseParallelRLCBranchLib/Three-Phase Parallel RLC Branch  LConnTagsString=A|B|C  RConnTagsString=A|B|C  BranchType=RLC  Resistance=(0.26874)*Zbase  Inductance=(0.56208)*Zbase/Wbase  Capacitance=(0.2685)*Ybase/Wbase  Measurements=None
  Branch67-68 : spsThreePhaseSeriesRLCBranchLib/Three-Phase Series RLC Branch  LConnTagsString=A|B|C  RConnTagsString=A|B|C  BranchType=RL  Resistance=(0.0009)*Zbase  Inductance=(0.0094)*Zbase/Wbase  Capacitance=1e-6  Measurements=None
  Branch68-68 : spsThreePhaseParallelRLCBranchLib/Three-Phase Parallel RLC Branch  LConnTagsString=A|B|C  RConnTagsString=A|B|C  BranchType=RLC  Resistance=(0.2735)*Zbase  Inductance=(2.8119)*Zbase/Wbase  Capacitance=(0.466)*Ybase/Wbase  Measurements=None
  Branch7-23 : spsThreePhaseSeriesRLCBranchLib/Three-Phase Series RLC Branch  LConnTagsString=A|B|C  RConnTagsString=A|B|C  BranchType=RL  Resistance=(0.0005)*Zbase  Inductance=(0.0272)*Zbase/Wbase  Capacitance=1e-6  Measurements=None
  Branch7-7 : spsThreePhaseParallelRLCBranchLib/Three-Phase Parallel RLC Branch  LConnTagsString=A|B|C  RConnTagsString=A|B|C  BranchType=C  Resistance=(Inf)*Zbase  Inductance=(Inf)*Zbase/Wbase  Capacitance=(5e-08)*Ybase/Wbase  Measurements=None
  Branch8-25 : spsThreePhaseSeriesRLCBranchLib/Three-Phase Series RLC Branch  LConnTagsString=A|B|C  RConnTagsString=A|B|C  BranchType=RL  Resistance=(0.0006)*Zbase  Inductance=(0.0232)*Zbase/Wbase  Capacitance=1e-6  Measurements=None
  Branch8-8 : spsThreePhaseParallelRLCBranchLib/Three-Phase Parallel RLC Branch  LConnTagsString=A|B|C  RConnTagsString=A|B|C  BranchType=C  Resistance=(Inf)*Zbase  Inductance=(Inf)*Zbase/Wbase  Capacitance=(5e-08)*Ybase/Wbase  Measurements=None
  Branch9-29 : spsThreePhaseSeriesRLCBranchLib/Three-Phase Series RLC Branch  LConnTagsString=A|B|C  RConnTagsString=A|B|C  BranchType=RL  Resistance=(0.0008)*Zbase  Inductance=(0.0156)*Zbase/Wbase  Capacitance=1e-6  Measurements=None
  Branch9-9 : spsThreePhaseParallelRLCBranchLib/Three-Phase Parallel RLC Branch  LConnTagsString=A|B|C  RConnTagsString=A|B|C  BranchType=C  Resistance=(Inf)*Zbase  Inductance=(Inf)*Zbase/Wbase  Capacitance=(5e-08)*Ybase/Wbase  Measurements=None
  Bus{1..68} (68 alike) : SimplusGT/Three-Phase Bus  Vbase=1  Sbase=1
      settings: SourceProductName=Simplus Grid Tool
  D-GND{1..17,26..29,35,39,43..45,50..51,58..59} (30 alike) : spsGroundLib/Ground  LConnTagsString=a
  D-Scope{1..17,26..29,35,39,43..45,50..51,58..59} (30 alike) : Scope  NumInputPorts=7
  DS-Bus{1..17,26..29,35,39,43..45,50..51,58..59} (30 alike) : BusSelector  OutputSignals=v_dq,i_dq,v_abc,i_abc,w,theta,pq
  SM_8th_AVRPSSGOV10 : SimplusGT/SynchronousMachineFull_SMAVRPSSGOV (dq-Frame System Object)  Ts=Ts  Sbase=Sbase  Vbase=Vbase  Wbase=Wbase  ApparatusType=ApparatusType{10}  ApparatusPara=ApparatusPara{10}  PowerFlow=ApparatusPowerFlow{10}  x0=x_e{10}  OtherInputs=OtherInputs{10}  DiscreMethod=Hybrid Trapezoidal  EnableInsideModification=off  DiscreDampingFlag=on  DiscreDampingValue=ApparatusDiscreDamping{10}  LinearizationTimes=1  DirectFeedthrough=off
      settings: SourceProductName=Simplus Grid Tool
  SM_8th_AVRPSSGOV11 : SimplusGT/SynchronousMachineFull_SMAVRPSSGOV (dq-Frame System Object)  Ts=Ts  Sbase=Sbase  Vbase=Vbase  Wbase=Wbase  ApparatusType=ApparatusType{11}  ApparatusPara=ApparatusPara{11}  PowerFlow=ApparatusPowerFlow{11}  x0=x_e{11}  OtherInputs=OtherInputs{11}  DiscreMethod=Hybrid Trapezoidal  EnableInsideModification=off  DiscreDampingFlag=on  DiscreDampingValue=ApparatusDiscreDamping{11}  LinearizationTimes=1  DirectFeedthrough=off
      settings: SourceProductName=Simplus Grid Tool
  SM_8th_AVRPSSGOV12 : SimplusGT/SynchronousMachineFull_SMAVRPSSGOV (dq-Frame System Object)  Ts=Ts  Sbase=Sbase  Vbase=Vbase  Wbase=Wbase  ApparatusType=ApparatusType{12}  ApparatusPara=ApparatusPara{12}  PowerFlow=ApparatusPowerFlow{12}  x0=x_e{12}  OtherInputs=OtherInputs{12}  DiscreMethod=Hybrid Trapezoidal  EnableInsideModification=off  DiscreDampingFlag=on  DiscreDampingValue=ApparatusDiscreDamping{12}  LinearizationTimes=1  DirectFeedthrough=off
      settings: SourceProductName=Simplus Grid Tool
  SM_8th_AVRPSSGOV16 : SimplusGT/SynchronousMachineFull_SMAVRPSSGOV (dq-Frame System Object)  Ts=Ts  Sbase=Sbase  Vbase=Vbase  Wbase=Wbase  ApparatusType=ApparatusType{16}  ApparatusPara=ApparatusPara{16}  PowerFlow=ApparatusPowerFlow{16}  x0=x_e{16}  OtherInputs=OtherInputs{16}  DiscreMethod=Hybrid Trapezoidal  EnableInsideModification=off  DiscreDampingFlag=on  DiscreDampingValue=ApparatusDiscreDamping{16}  LinearizationTimes=1  DirectFeedthrough=off
      settings: SourceProductName=Simplus Grid Tool
  SM_8th_AVRPSSGOV2 : SimplusGT/SynchronousMachineFull_SMAVRPSSGOV (dq-Frame System Object)  Ts=Ts  Sbase=Sbase  Vbase=Vbase  Wbase=Wbase  ApparatusType=ApparatusType{2}  ApparatusPara=ApparatusPara{2}  PowerFlow=ApparatusPowerFlow{2}  x0=x_e{2}  OtherInputs=OtherInputs{2}  DiscreMethod=Hybrid Trapezoidal  EnableInsideModification=off  DiscreDampingFlag=on  DiscreDampingValue=ApparatusDiscreDamping{2}  LinearizationTimes=1  DirectFeedthrough=off
      settings: SourceProductName=Simplus Grid Tool
  SM_8th_AVRPSSGOV3 : SimplusGT/SynchronousMachineFull_SMAVRPSSGOV (dq-Frame System Object)  Ts=Ts  Sbase=Sbase  Vbase=Vbase  Wbase=Wbase  ApparatusType=ApparatusType{3}  ApparatusPara=ApparatusPara{3}  PowerFlow=ApparatusPowerFlow{3}  x0=x_e{3}  OtherInputs=OtherInputs{3}  DiscreMethod=Hybrid Trapezoidal  EnableInsideModification=off  DiscreDampingFlag=on  DiscreDampingValue=ApparatusDiscreDamping{3}  LinearizationTimes=1  DirectFeedthrough=off
      settings: SourceProductName=Simplus Grid Tool
  SM_8th_AVRPSSGOV4 : SimplusGT/SynchronousMachineFull_SMAVRPSSGOV (dq-Frame System Object)  Ts=Ts  Sbase=Sbase  Vbase=Vbase  Wbase=Wbase  ApparatusType=ApparatusType{4}  ApparatusPara=ApparatusPara{4}  PowerFlow=ApparatusPowerFlow{4}  x0=x_e{4}  OtherInputs=OtherInputs{4}  DiscreMethod=Hybrid Trapezoidal  EnableInsideModification=off  DiscreDampingFlag=on  DiscreDampingValue=ApparatusDiscreDamping{4}  LinearizationTimes=1  DirectFeedthrough=off
      settings: SourceProductName=Simplus Grid Tool
  SM_8th_AVRPSSGOV5 : SimplusGT/SynchronousMachineFull_SMAVRPSSGOV (dq-Frame System Object)  Ts=Ts  Sbase=Sbase  Vbase=Vbase  Wbase=Wbase  ApparatusType=ApparatusType{5}  ApparatusPara=ApparatusPara{5}  PowerFlow=ApparatusPowerFlow{5}  x0=x_e{5}  OtherInputs=OtherInputs{5}  DiscreMethod=Hybrid Trapezoidal  EnableInsideModification=off  DiscreDampingFlag=on  DiscreDampingValue=ApparatusDiscreDamping{5}  LinearizationTimes=1  DirectFeedthrough=off
      settings: SourceProductName=Simplus Grid Tool
  SM_8th_AVRPSSGOV6 : SimplusGT/SynchronousMachineFull_SMAVRPSSGOV (dq-Frame System Object)  Ts=Ts  Sbase=Sbase  Vbase=Vbase  Wbase=Wbase  ApparatusType=ApparatusType{6}  ApparatusPara=ApparatusPara{6}  PowerFlow=ApparatusPowerFlow{6}  x0=x_e{6}  OtherInputs=OtherInputs{6}  DiscreMethod=Hybrid Trapezoidal  EnableInsideModification=off  DiscreDampingFlag=on  DiscreDampingValue=ApparatusDiscreDamping{6}  LinearizationTimes=1  DirectFeedthrough=off
      settings: SourceProductName=Simplus Grid Tool
  SM_8th_AVRPSSGOV7 : SimplusGT/SynchronousMachineFull_SMAVRPSSGOV (dq-Frame System Object)  Ts=Ts  Sbase=Sbase  Vbase=Vbase  Wbase=Wbase  ApparatusType=ApparatusType{7}  ApparatusPara=ApparatusPara{7}  PowerFlow=ApparatusPowerFlow{7}  x0=x_e{7}  OtherInputs=OtherInputs{7}  DiscreMethod=Hybrid Trapezoidal  EnableInsideModification=off  DiscreDampingFlag=on  DiscreDampingValue=ApparatusDiscreDamping{7}  LinearizationTimes=1  DirectFeedthrough=off
      settings: SourceProductName=Simplus Grid Tool
  SM_8th_AVRPSSGOV8 : SimplusGT/SynchronousMachineFull_SMAVRPSSGOV (dq-Frame System Object)  Ts=Ts  Sbase=Sbase  Vbase=Vbase  Wbase=Wbase  ApparatusType=ApparatusType{8}  ApparatusPara=ApparatusPara{8}  PowerFlow=ApparatusPowerFlow{8}  x0=x_e{8}  OtherInputs=OtherInputs{8}  DiscreMethod=Hybrid Trapezoidal  EnableInsideModification=off  DiscreDampingFlag=on  DiscreDampingValue=ApparatusDiscreDamping{8}  LinearizationTimes=1  DirectFeedthrough=off
      settings: SourceProductName=Simplus Grid Tool
  SM_8th_AVRPSSGOV9 : SimplusGT/SynchronousMachineFull_SMAVRPSSGOV (dq-Frame System Object)  Ts=Ts  Sbase=Sbase  Vbase=Vbase  Wbase=Wbase  ApparatusType=ApparatusType{9}  ApparatusPara=ApparatusPara{9}  PowerFlow=ApparatusPowerFlow{9}  x0=x_e{9}  OtherInputs=OtherInputs{9}  DiscreMethod=Hybrid Trapezoidal  EnableInsideModification=off  DiscreDampingFlag=on  DiscreDampingValue=ApparatusDiscreDamping{9}  LinearizationTimes=1  DirectFeedthrough=off
      settings: SourceProductName=Simplus Grid Tool
  SM_8th_GOV1 : SimplusGT/SynchronousMachineFull_SM_GOV (dq-Frame System Object)  Ts=Ts  Sbase=Sbase  Vbase=Vbase  Wbase=Wbase  ApparatusType=ApparatusType{1}  ApparatusPara=ApparatusPara{1}  PowerFlow=ApparatusPowerFlow{1}  x0=x_e{1}  OtherInputs=OtherInputs{1}  DiscreMethod=Hybrid Trapezoidal  EnableInsideModification=off  DiscreDampingFlag=on  DiscreDampingValue=ApparatusDiscreDamping{1}  LinearizationTimes=1  DirectFeedthrough=off
      settings: SourceProductName=Simplus Grid Tool
  SM_8th_GOV13 : SimplusGT/SynchronousMachineFull_SM_GOV (dq-Frame System Object)  Ts=Ts  Sbase=Sbase  Vbase=Vbase  Wbase=Wbase  ApparatusType=ApparatusType{13}  ApparatusPara=ApparatusPara{13}  PowerFlow=ApparatusPowerFlow{13}  x0=x_e{13}  OtherInputs=OtherInputs{13}  DiscreMethod=Hybrid Trapezoidal  EnableInsideModification=off  DiscreDampingFlag=on  DiscreDampingValue=ApparatusDiscreDamping{13}  LinearizationTimes=1  DirectFeedthrough=off
      settings: SourceProductName=Simplus Grid Tool
  SM_8th_GOV14 : SimplusGT/SynchronousMachineFull_SM_GOV (dq-Frame System Object)  Ts=Ts  Sbase=Sbase  Vbase=Vbase  Wbase=Wbase  ApparatusType=ApparatusType{14}  ApparatusPara=ApparatusPara{14}  PowerFlow=ApparatusPowerFlow{14}  x0=x_e{14}  OtherInputs=OtherInputs{14}  DiscreMethod=Hybrid Trapezoidal  EnableInsideModification=off  DiscreDampingFlag=on  DiscreDampingValue=ApparatusDiscreDamping{14}  LinearizationTimes=1  DirectFeedthrough=off
      settings: SourceProductName=Simplus Grid Tool
  SM_8th_GOV15 : SimplusGT/SynchronousMachineFull_SM_GOV (dq-Frame System Object)  Ts=Ts  Sbase=Sbase  Vbase=Vbase  Wbase=Wbase  ApparatusType=ApparatusType{15}  ApparatusPara=ApparatusPara{15}  PowerFlow=ApparatusPowerFlow{15}  x0=x_e{15}  OtherInputs=OtherInputs{15}  DiscreMethod=Hybrid Trapezoidal  EnableInsideModification=off  DiscreDampingFlag=on  DiscreDampingValue=ApparatusDiscreDamping{15}  LinearizationTimes=1  DirectFeedthrough=off
      settings: SourceProductName=Simplus Grid Tool
  Three-Phase Breaker : spsThreePhaseBreakerLib/Three-Phase Breaker  InitialState=open  SwitchA=on  SwitchB=on  SwitchC=on  SwitchTimes=[16]  External=off  BreakerResistance=0.01  SnubberResistance=1e6  SnubberCapacitance=inf  Measurements=None
  Three-Phase Breaker1 : spsThreePhaseBreakerLib/Three-Phase Breaker  InitialState=open  SwitchA=on  SwitchB=on  SwitchC=on  SwitchTimes=[16]  External=off  BreakerResistance=0.01  SnubberResistance=1e6  SnubberCapacitance=inf  Measurements=None
  Three-Phase Breaker2 : spsThreePhaseBreakerLib/Three-Phase Breaker  InitialState=open  SwitchA=on  SwitchB=on  SwitchC=on  SwitchTimes=[160]  External=off  BreakerResistance=0.01  SnubberResistance=1e6  SnubberCapacitance=inf  Measurements=None
  Transformer10-31 : spsThreePhaseTransformerTwoWindingsLib/Three-Phase Transformer (Two Windings)  Winding1Connection=Yg  Winding2Connection=Yg  CoreType=Three single-phase transformers  SetSaturation=off  Hysteresis=off  DataFile='hysteresis'  SetInitialFlux=off  Measurements=None  UNITS=pu  NominalPower=[Sbase, Fbase]  Winding1=[1.04*Vbase, 0, 0]  Winding2=[Vbase, 0, 0]  Rm=1e4  Lm=1e4  L0=0.5  Saturation=[ 0,0 ; 0.0024,1.2 ; 1.0,1.52 ]  InitialFluxes=[ 0.8 , -0.8 , 0.7 ]  BreakLoop=off  DiscreteSolver=Trapezoidal iterative  DataType=off  TransfoNumber=1
  Transformer11-32 : spsThreePhaseTransformerTwoWindingsLib/Three-Phase Transformer (Two Windings)  Winding1Connection=Yg  Winding2Connection=Yg  CoreType=Three single-phase transformers  SetSaturation=off  Hysteresis=off  DataFile='hysteresis'  SetInitialFlux=off  Measurements=None  UNITS=pu  NominalPower=[Sbase, Fbase]  Winding1=[1.04*Vbase, 0, 0]  Winding2=[Vbase, 0, 0]  Rm=1e4  Lm=1e4  L0=0.5  Saturation=[ 0,0 ; 0.0024,1.2 ; 1.0,1.52 ]  InitialFluxes=[ 0.8 , -0.8 , 0.7 ]  BreakLoop=off  DiscreteSolver=Trapezoidal iterative  DataType=off  TransfoNumber=1
  Transformer12-36 : spsThreePhaseTransformerTwoWindingsLib/Three-Phase Transformer (Two Windings)  Winding1Connection=Yg  Winding2Connection=Yg  CoreType=Three single-phase transformers  SetSaturation=off  Hysteresis=off  DataFile='hysteresis'  SetInitialFlux=off  Measurements=None  UNITS=pu  NominalPower=[Sbase, Fbase]  Winding1=[1.04*Vbase, 0, 0]  Winding2=[Vbase, 0, 0]  Rm=1e4  Lm=1e4  L0=0.5  Saturation=[ 0,0 ; 0.0024,1.2 ; 1.0,1.52 ]  InitialFluxes=[ 0.8 , -0.8 , 0.7 ]  BreakLoop=off  DiscreteSolver=Trapezoidal iterative  DataType=off  TransfoNumber=1
  Transformer13-17 : spsThreePhaseTransformerTwoWindingsLib/Three-Phase Transformer (Two Windings)  Winding1Connection=Yg  Winding2Connection=Yg  CoreType=Three single-phase transformers  SetSaturation=off  Hysteresis=off  DataFile='hysteresis'  SetInitialFlux=off  Measurements=None  UNITS=pu  NominalPower=[Sbase, Fbase]  Winding1=[1.04*Vbase, 0, 0]  Winding2=[Vbase, 0, 0]  Rm=1e4  Lm=1e4  L0=0.5  Saturation=[ 0,0 ; 0.0024,1.2 ; 1.0,1.52 ]  InitialFluxes=[ 0.8 , -0.8 , 0.7 ]  BreakLoop=off  DiscreteSolver=Trapezoidal iterative  DataType=off  TransfoNumber=1
  Transformer16-54 : spsThreePhaseTransformerTwoWindingsLib/Three-Phase Transformer (Two Windings)  Winding1Connection=Yg  Winding2Connection=Yg  CoreType=Three single-phase transformers  SetSaturation=off  Hysteresis=off  DataFile='hysteresis'  SetInitialFlux=off  Measurements=None  UNITS=pu  NominalPower=[Sbase, Fbase]  Winding1=[1.025*Vbase, 0, 0]  Winding2=[Vbase, 0, 0]  Rm=1e4  Lm=1e4  L0=0.5  Saturation=[ 0,0 ; 0.0024,1.2 ; 1.0,1.52 ]  InitialFluxes=[ 0.8 , -0.8 , 0.7 ]  BreakLoop=off  DiscreteSolver=Trapezoidal iterative  DataType=off  TransfoNumber=1
  Transformer19-20 : spsThreePhaseTransformerTwoWindingsLib/Three-Phase Transformer (Two Windings)  Winding1Connection=Yg  Winding2Connection=Yg  CoreType=Three single-phase transformers  SetSaturation=off  Hysteresis=off  DataFile='hysteresis'  SetInitialFlux=off  Measurements=None  UNITS=pu  NominalPower=[Sbase, Fbase]  Winding1=[0.9434*Vbase, 0, 0]  Winding2=[Vbase, 0, 0]  Rm=1e4  Lm=1e4  L0=0.5  Saturation=[ 0,0 ; 0.0024,1.2 ; 1.0,1.52 ]  InitialFluxes=[ 0.8 , -0.8 , 0.7 ]  BreakLoop=off  DiscreteSolver=Trapezoidal iterative  DataType=off  TransfoNumber=1
  Transformer2-58 : spsThreePhaseTransformerTwoWindingsLib/Three-Phase Transformer (Two Windings)  Winding1Connection=Yg  Winding2Connection=Yg  CoreType=Three single-phase transformers  SetSaturation=off  Hysteresis=off  DataFile='hysteresis'  SetInitialFlux=off  Measurements=None  UNITS=pu  NominalPower=[Sbase, Fbase]  Winding1=[1.07*Vbase, 0, 0]  Winding2=[Vbase, 0, 0]  Rm=1e4  Lm=1e4  L0=0.5  Saturation=[ 0,0 ; 0.0024,1.2 ; 1.0,1.52 ]  InitialFluxes=[ 0.8 , -0.8 , 0.7 ]  BreakLoop=off  DiscreteSolver=Trapezoidal iterative  DataType=off  TransfoNumber=1
  Transformer3-62 : spsThreePhaseTransformerTwoWindingsLib/Three-Phase Transformer (Two Windings)  Winding1Connection=Yg  Winding2Connection=Yg  CoreType=Three single-phase transformers  SetSaturation=off  Hysteresis=off  DataFile='hysteresis'  SetInitialFlux=off  Measurements=None  UNITS=pu  NominalPower=[Sbase, Fbase]  Winding1=[1.07*Vbase, 0, 0]  Winding2=[Vbase, 0, 0]  Rm=1e4  Lm=1e4  L0=0.5  Saturation=[ 0,0 ; 0.0024,1.2 ; 1.0,1.52 ]  InitialFluxes=[ 0.8 , -0.8 , 0.7 ]  BreakLoop=off  DiscreteSolver=Trapezoidal iterative  DataType=off  TransfoNumber=1
  Transformer34-35 : spsThreePhaseTransformerTwoWindingsLib/Three-Phase Transformer (Two Windings)  Winding1Connection=Yg  Winding2Connection=Yg  CoreType=Three single-phase transformers  SetSaturation=off  Hysteresis=off  DataFile='hysteresis'  SetInitialFlux=off  Measurements=None  UNITS=pu  NominalPower=[Sbase, Fbase]  Winding1=[0.946*Vbase, 0, 0]  Winding2=[Vbase, 0, 0]  Rm=1e4  Lm=1e4  L0=0.5  Saturation=[ 0,0 ; 0.0024,1.2 ; 1.0,1.52 ]  InitialFluxes=[ 0.8 , -0.8 , 0.7 ]  BreakLoop=off  DiscreteSolver=Trapezoidal iterative  DataType=off  TransfoNumber=1
  Transformer4-19 : spsThreePhaseTransformerTwoWindingsLib/Three-Phase Transformer (Two Windings)  Winding1Connection=Yg  Winding2Connection=Yg  CoreType=Three single-phase transformers  SetSaturation=off  Hysteresis=off  DataFile='hysteresis'  SetInitialFlux=off  Measurements=None  UNITS=pu  NominalPower=[Sbase, Fbase]  Winding1=[1.07*Vbase, 0, 0]  Winding2=[Vbase, 0, 0]  Rm=1e4  Lm=1e4  L0=0.5  Saturation=[ 0,0 ; 0.0024,1.2 ; 1.0,1.52 ]  InitialFluxes=[ 0.8 , -0.8 , 0.7 ]  BreakLoop=off  DiscreteSolver=Trapezoidal iterative  DataType=off  TransfoNumber=1
  Transformer5-20 : spsThreePhaseTransformerTwoWindingsLib/Three-Phase Transformer (Two Windings)  Winding1Connection=Yg  Winding2Connection=Yg  CoreType=Three single-phase transformers  SetSaturation=off  Hysteresis=off  DataFile='hysteresis'  SetInitialFlux=off  Measurements=None  UNITS=pu  NominalPower=[Sbase, Fbase]  Winding1=[1.009*Vbase, 0, 0]  Winding2=[Vbase, 0, 0]  Rm=1e4  Lm=1e4  L0=0.5  Saturation=[ 0,0 ; 0.0024,1.2 ; 1.0,1.52 ]  InitialFluxes=[ 0.8 , -0.8 , 0.7 ]  BreakLoop=off  DiscreteSolver=Trapezoidal iterative  DataType=off  TransfoNumber=1
  Transformer6-22 : spsThreePhaseTransformerTwoWindingsLib/Three-Phase Transformer (Two Windings)  Winding1Connection=Yg  Winding2Connection=Yg  CoreType=Three single-phase transformers  SetSaturation=off  Hysteresis=off  DataFile='hysteresis'  SetInitialFlux=off  Measurements=None  UNITS=pu  NominalPower=[Sbase, Fbase]  Winding1=[1.025*Vbase, 0, 0]  Winding2=[Vbase, 0, 0]  Rm=1e4  Lm=1e4  L0=0.5  Saturation=[ 0,0 ; 0.0024,1.2 ; 1.0,1.52 ]  InitialFluxes=[ 0.8 , -0.8 , 0.7 ]  BreakLoop=off  DiscreteSolver=Trapezoidal iterative  DataType=off  TransfoNumber=1
  Transformer63-64 : spsThreePhaseTransformerTwoWindingsLib/Three-Phase Transformer (Two Windings)  Winding1Connection=Yg  Winding2Connection=Yg  CoreType=Three single-phase transformers  SetSaturation=off  Hysteresis=off  DataFile='hysteresis'  SetInitialFlux=off  Measurements=None  UNITS=pu  NominalPower=[Sbase, Fbase]  Winding1=[1.06*Vbase, 0, 0]  Winding2=[Vbase, 0, 0]  Rm=1e4  Lm=1e4  L0=0.5  Saturation=[ 0,0 ; 0.0024,1.2 ; 1.0,1.52 ]  InitialFluxes=[ 0.8 , -0.8 , 0.7 ]  BreakLoop=off  DiscreteSolver=Trapezoidal iterative  DataType=off  TransfoNumber=1
  Transformer64-65 : spsThreePhaseTransformerTwoWindingsLib/Three-Phase Transformer (Two Windings)  Winding1Connection=Yg  Winding2Connection=Yg  CoreType=Three single-phase transformers  SetSaturation=off  Hysteresis=off  DataFile='hysteresis'  SetInitialFlux=off  Measurements=None  UNITS=pu  NominalPower=[Sbase, Fbase]  Winding1=[0.9434*Vbase, 0, 0]  Winding2=[Vbase, 0, 0]  Rm=1e4  Lm=1e4  L0=0.5  Saturation=[ 0,0 ; 0.0024,1.2 ; 1.0,1.52 ]  InitialFluxes=[ 0.8 , -0.8 , 0.7 ]  BreakLoop=off  DiscreteSolver=Trapezoidal iterative  DataType=off  TransfoNumber=1
  Transformer8-25 : spsThreePhaseTransformerTwoWindingsLib/Three-Phase Transformer (Two Windings)  Winding1Connection=Yg  Winding2Connection=Yg  CoreType=Three single-phase transformers  SetSaturation=off  Hysteresis=off  DataFile='hysteresis'  SetInitialFlux=off  Measurements=None  UNITS=pu  NominalPower=[Sbase, Fbase]  Winding1=[1.025*Vbase, 0, 0]  Winding2=[Vbase, 0, 0]  Rm=1e4  Lm=1e4  L0=0.5  Saturation=[ 0,0 ; 0.0024,1.2 ; 1.0,1.52 ]  InitialFluxes=[ 0.8 , -0.8 , 0.7 ]  BreakLoop=off  DiscreteSolver=Trapezoidal iterative  DataType=off  TransfoNumber=1
  Transformer9-29 : spsThreePhaseTransformerTwoWindingsLib/Three-Phase Transformer (Two Windings)  Winding1Connection=Yg  Winding2Connection=Yg  CoreType=Three single-phase transformers  SetSaturation=off  Hysteresis=off  DataFile='hysteresis'  SetInitialFlux=off  Measurements=None  UNITS=pu  NominalPower=[Sbase, Fbase]  Winding1=[1.025*Vbase, 0, 0]  Winding2=[Vbase, 0, 0]  Rm=1e4  Lm=1e4  L0=0.5  Saturation=[ 0,0 ; 0.0024,1.2 ; 1.0,1.52 ]  InitialFluxes=[ 0.8 , -0.8 , 0.7 ]  BreakLoop=off  DiscreteSolver=Trapezoidal iterative  DataType=off  TransfoNumber=1
  VSI-PLL17 : SimplusGT/Grid-Following Voltage-Source Inverter (dq-Frame System Object)_old  Ts=Ts  Sbase=Sbase  Vbase=Vbase  Wbase=Wbase  ApparatusType=ApparatusType{17}  ApparatusPara=ApparatusPara{17}  PowerFlow=ApparatusPowerFlow{17}  x0=x_e{17}  OtherInputs=OtherInputs{17}  DiscreMethod=Hybrid Trapezoidal  EnableInsideModification=off  DiscreDampingFlag=on  DiscreDampingValue=ApparatusDiscreDamping{17}  LinearizationTimes=1  DirectFeedthrough=off
      settings: SourceProductName=Simplus Grid Tool
  VSI-PLL26 : SimplusGT/Grid-Following Voltage-Source Inverter (dq-Frame System Object)_old  Ts=Ts  Sbase=Sbase  Vbase=Vbase  Wbase=Wbase  ApparatusType=ApparatusType{26}  ApparatusPara=ApparatusPara{26}  PowerFlow=ApparatusPowerFlow{26}  x0=x_e{26}  OtherInputs=OtherInputs{26}  DiscreMethod=Hybrid Trapezoidal  EnableInsideModification=off  DiscreDampingFlag=on  DiscreDampingValue=ApparatusDiscreDamping{26}  LinearizationTimes=1  DirectFeedthrough=off
      settings: SourceProductName=Simplus Grid Tool
  VSI-PLL27 : SimplusGT/Grid-Following Voltage-Source Inverter (dq-Frame System Object)_old  Ts=Ts  Sbase=Sbase  Vbase=Vbase  Wbase=Wbase  ApparatusType=ApparatusType{27}  ApparatusPara=ApparatusPara{27}  PowerFlow=ApparatusPowerFlow{27}  x0=x_e{27}  OtherInputs=OtherInputs{27}  DiscreMethod=Hybrid Trapezoidal  EnableInsideModification=off  DiscreDampingFlag=on  DiscreDampingValue=ApparatusDiscreDamping{27}  LinearizationTimes=1  DirectFeedthrough=off
      settings: SourceProductName=Simplus Grid Tool
  VSI-PLL28 : SimplusGT/Grid-Following Voltage-Source Inverter (dq-Frame System Object)_old  Ts=Ts  Sbase=Sbase  Vbase=Vbase  Wbase=Wbase  ApparatusType=ApparatusType{28}  ApparatusPara=ApparatusPara{28}  PowerFlow=ApparatusPowerFlow{28}  x0=x_e{28}  OtherInputs=OtherInputs{28}  DiscreMethod=Hybrid Trapezoidal  EnableInsideModification=off  DiscreDampingFlag=on  DiscreDampingValue=ApparatusDiscreDamping{28}  LinearizationTimes=1  DirectFeedthrough=off
      settings: SourceProductName=Simplus Grid Tool
  VSI-PLL29 : SimplusGT/Grid-Following Voltage-Source Inverter (dq-Frame System Object)_old  Ts=Ts  Sbase=Sbase  Vbase=Vbase  Wbase=Wbase  ApparatusType=ApparatusType{29}  ApparatusPara=ApparatusPara{29}  PowerFlow=ApparatusPowerFlow{29}  x0=x_e{29}  OtherInputs=OtherInputs{29}  DiscreMethod=Hybrid Trapezoidal  EnableInsideModification=off  DiscreDampingFlag=on  DiscreDampingValue=ApparatusDiscreDamping{29}  LinearizationTimes=1  DirectFeedthrough=off
      settings: SourceProductName=Simplus Grid Tool
  VSI-PLL35 : SimplusGT/Grid-Following Voltage-Source Inverter (dq-Frame System Object)_old  Ts=Ts  Sbase=Sbase  Vbase=Vbase  Wbase=Wbase  ApparatusType=ApparatusType{35}  ApparatusPara=ApparatusPara{35}  PowerFlow=ApparatusPowerFlow{35}  x0=x_e{35}  OtherInputs=OtherInputs{35}  DiscreMethod=Hybrid Trapezoidal  EnableInsideModification=off  DiscreDampingFlag=on  DiscreDampingValue=ApparatusDiscreDamping{35}  LinearizationTimes=1  DirectFeedthrough=off
      settings: SourceProductName=Simplus Grid Tool
  VSI-PLL39 : SimplusGT/Grid-Following Voltage-Source Inverter (dq-Frame System Object)_old  Ts=Ts  Sbase=Sbase  Vbase=Vbase  Wbase=Wbase  ApparatusType=ApparatusType{39}  ApparatusPara=ApparatusPara{39}  PowerFlow=ApparatusPowerFlow{39}  x0=x_e{39}  OtherInputs=OtherInputs{39}  DiscreMethod=Hybrid Trapezoidal  EnableInsideModification=off  DiscreDampingFlag=on  DiscreDampingValue=ApparatusDiscreDamping{39}  LinearizationTimes=1  DirectFeedthrough=off
      settings: SourceProductName=Simplus Grid Tool
  VSI-PLL43 : SimplusGT/Grid-Following Voltage-Source Inverter (dq-Frame System Object)_old  Ts=Ts  Sbase=Sbase  Vbase=Vbase  Wbase=Wbase  ApparatusType=ApparatusType{43}  ApparatusPara=ApparatusPara{43}  PowerFlow=ApparatusPowerFlow{43}  x0=x_e{43}  OtherInputs=OtherInputs{43}  DiscreMethod=Hybrid Trapezoidal  EnableInsideModification=off  DiscreDampingFlag=on  DiscreDampingValue=ApparatusDiscreDamping{43}  LinearizationTimes=1  DirectFeedthrough=off
      settings: SourceProductName=Simplus Grid Tool
  VSI-PLL44 : SimplusGT/Grid-Following Voltage-Source Inverter (dq-Frame System Object)_old  Ts=Ts  Sbase=Sbase  Vbase=Vbase  Wbase=Wbase  ApparatusType=ApparatusType{44}  ApparatusPara=ApparatusPara{44}  PowerFlow=ApparatusPowerFlow{44}  x0=x_e{44}  OtherInputs=OtherInputs{44}  DiscreMethod=Hybrid Trapezoidal  EnableInsideModification=off  DiscreDampingFlag=on  DiscreDampingValue=ApparatusDiscreDamping{44}  LinearizationTimes=1  DirectFeedthrough=off
      settings: SourceProductName=Simplus Grid Tool
  VSI-PLL45 : SimplusGT/Grid-Following Voltage-Source Inverter (dq-Frame System Object)_old  Ts=Ts  Sbase=Sbase  Vbase=Vbase  Wbase=Wbase  ApparatusType=ApparatusType{45}  ApparatusPara=ApparatusPara{45}  PowerFlow=ApparatusPowerFlow{45}  x0=x_e{45}  OtherInputs=OtherInputs{45}  DiscreMethod=Hybrid Trapezoidal  EnableInsideModification=off  DiscreDampingFlag=on  DiscreDampingValue=ApparatusDiscreDamping{45}  LinearizationTimes=1  DirectFeedthrough=off
      settings: SourceProductName=Simplus Grid Tool
  VSI-PLL50 : SimplusGT/Grid-Following Voltage-Source Inverter (dq-Frame System Object)_old  Ts=Ts  Sbase=Sbase  Vbase=Vbase  Wbase=Wbase  ApparatusType=ApparatusType{50}  ApparatusPara=ApparatusPara{50}  PowerFlow=ApparatusPowerFlow{50}  x0=x_e{50}  OtherInputs=OtherInputs{50}  DiscreMethod=Hybrid Trapezoidal  EnableInsideModification=off  DiscreDampingFlag=on  DiscreDampingValue=ApparatusDiscreDamping{50}  LinearizationTimes=1  DirectFeedthrough=off
      settings: SourceProductName=Simplus Grid Tool
  VSI-PLL51 : SimplusGT/Grid-Following Voltage-Source Inverter (dq-Frame System Object)_old  Ts=Ts  Sbase=Sbase  Vbase=Vbase  Wbase=Wbase  ApparatusType=ApparatusType{51}  ApparatusPara=ApparatusPara{51}  PowerFlow=ApparatusPowerFlow{51}  x0=x_e{51}  OtherInputs=OtherInputs{51}  DiscreMethod=Hybrid Trapezoidal  EnableInsideModification=off  DiscreDampingFlag=on  DiscreDampingValue=ApparatusDiscreDamping{51}  LinearizationTimes=1  DirectFeedthrough=off
      settings: SourceProductName=Simplus Grid Tool
  VSI-PLL58 : SimplusGT/Grid-Following Voltage-Source Inverter (dq-Frame System Object)_old  Ts=Ts  Sbase=Sbase  Vbase=Vbase  Wbase=Wbase  ApparatusType=ApparatusType{58}  ApparatusPara=ApparatusPara{58}  PowerFlow=ApparatusPowerFlow{58}  x0=x_e{58}  OtherInputs=OtherInputs{58}  DiscreMethod=Hybrid Trapezoidal  EnableInsideModification=off  DiscreDampingFlag=on  DiscreDampingValue=ApparatusDiscreDamping{58}  LinearizationTimes=1  DirectFeedthrough=off
      settings: SourceProductName=Simplus Grid Tool
  VSI-PLL59 : SimplusGT/Grid-Following Voltage-Source Inverter (dq-Frame System Object)_old  Ts=Ts  Sbase=Sbase  Vbase=Vbase  Wbase=Wbase  ApparatusType=ApparatusType{59}  ApparatusPara=ApparatusPara{59}  PowerFlow=ApparatusPowerFlow{59}  x0=x_e{59}  OtherInputs=OtherInputs{59}  DiscreMethod=Hybrid Trapezoidal  EnableInsideModification=off  DiscreDampingFlag=on  DiscreDampingValue=ApparatusDiscreDamping{59}  LinearizationTimes=1  DirectFeedthrough=off
      settings: SourceProductName=Simplus Grid Tool
  powergui : sps_lib/powergui  Priority=1  SimulationMode=Discrete  SampleTime=Ts  frequency=60  Iterations=50  frequencyindice=0  Pbase=100e6  ErrMax=1e-4  UnitsV=kV  UnitsW=MW  buscounter=0  FunctionMessages=off  echomessages=off  EnableUseOfTLC=off  CurrentSourceSwitches=off  DisableSnubberDevices=off  DisableRonSwitches=off  DisableVfSwitches=off  DisplayEquations=off  AutomaticDiscreteSolvers=off  SolverType=Tustin/Backward Euler (TBE)  Interpol=off  ExternalGateDelay=off  methode=off  Ts=100  x0status=blocks  SPID=on  SwTol=0  HookPort=off  NonlinearTolerance=1e-4  nMaxIteration=100  ContinueOnMaxIteration=off  RestoreLinks=warning  ResistiveCurrentMeasurement=off  Frange=[0:2:500]  Ylog=off  Xlog=on  ShowGrid=off  save=off  variable=ZData  structure=0  ZoomFFT=off  StartTime=0.0  cycles=1  DisplayStyle=1  fundamental=60  FreqAxis=off  MaxFrequency=1000  frequencyindicesteady=1  RmsSteady=1  display=off
  wires:
  SM_8th_GOV1/1 -> DS-Bus1/1
  DS-Bus1/1 -> D-Scope1/1  "<v_dq>"
  DS-Bus1/2 -> D-Scope1/2  "<i_dq>"
  DS-Bus1/3 -> D-Scope1/3  "<v_abc>"
  DS-Bus1/4 -> D-Scope1/4  "<i_abc>"
  DS-Bus1/5 -> D-Scope1/5  "<w>"
  DS-Bus1/6 -> D-Scope1/6  "<theta>"
  DS-Bus1/7 -> D-Scope1/7  "<pq>"
  SM_8th_AVRPSSGOV2/1 -> DS-Bus2/1
  DS-Bus2/1 -> D-Scope2/1  "<v_dq>"
  DS-Bus2/2 -> D-Scope2/2  "<i_dq>"
  DS-Bus2/3 -> D-Scope2/3  "<v_abc>"
  DS-Bus2/4 -> D-Scope2/4  "<i_abc>"
  DS-Bus2/5 -> D-Scope2/5  "<w>"
  DS-Bus2/6 -> D-Scope2/6  "<theta>"
  DS-Bus2/7 -> D-Scope2/7  "<pq>"
  SM_8th_AVRPSSGOV3/1 -> DS-Bus3/1
  DS-Bus3/1 -> D-Scope3/1  "<v_dq>"
  DS-Bus3/2 -> D-Scope3/2  "<i_dq>"
  DS-Bus3/3 -> D-Scope3/3  "<v_abc>"
  DS-Bus3/4 -> D-Scope3/4  "<i_abc>"
  DS-Bus3/5 -> D-Scope3/5  "<w>"
  DS-Bus3/6 -> D-Scope3/6  "<theta>"
  DS-Bus3/7 -> D-Scope3/7  "<pq>"
  SM_8th_AVRPSSGOV4/1 -> DS-Bus4/1
  DS-Bus4/1 -> D-Scope4/1  "<v_dq>"
  DS-Bus4/2 -> D-Scope4/2  "<i_dq>"
  DS-Bus4/3 -> D-Scope4/3  "<v_abc>"
  DS-Bus4/4 -> D-Scope4/4  "<i_abc>"
  DS-Bus4/5 -> D-Scope4/5  "<w>"
  DS-Bus4/6 -> D-Scope4/6  "<theta>"
  DS-Bus4/7 -> D-Scope4/7  "<pq>"
  SM_8th_AVRPSSGOV5/1 -> DS-Bus5/1
  DS-Bus5/1 -> D-Scope5/1  "<v_dq>"
  DS-Bus5/2 -> D-Scope5/2  "<i_dq>"
  DS-Bus5/3 -> D-Scope5/3  "<v_abc>"
  DS-Bus5/4 -> D-Scope5/4  "<i_abc>"
  DS-Bus5/5 -> D-Scope5/5  "<w>"
  DS-Bus5/6 -> D-Scope5/6  "<theta>"
  DS-Bus5/7 -> D-Scope5/7  "<pq>"
  SM_8th_AVRPSSGOV6/1 -> DS-Bus6/1
  DS-Bus6/1 -> D-Scope6/1  "<v_dq>"
  DS-Bus6/2 -> D-Scope6/2  "<i_dq>"
  DS-Bus6/3 -> D-Scope6/3  "<v_abc>"
  DS-Bus6/4 -> D-Scope6/4  "<i_abc>"
  DS-Bus6/5 -> D-Scope6/5  "<w>"
  DS-Bus6/6 -> D-Scope6/6  "<theta>"
  DS-Bus6/7 -> D-Scope6/7  "<pq>"
  SM_8th_AVRPSSGOV7/1 -> DS-Bus7/1
  DS-Bus7/1 -> D-Scope7/1  "<v_dq>"
  DS-Bus7/2 -> D-Scope7/2  "<i_dq>"
  DS-Bus7/3 -> D-Scope7/3  "<v_abc>"
  DS-Bus7/4 -> D-Scope7/4  "<i_abc>"
  DS-Bus7/5 -> D-Scope7/5  "<w>"
  DS-Bus7/6 -> D-Scope7/6  "<theta>"
  DS-Bus7/7 -> D-Scope7/7  "<pq>"
  SM_8th_AVRPSSGOV8/1 -> DS-Bus8/1
  DS-Bus8/1 -> D-Scope8/1  "<v_dq>"
  DS-Bus8/2 -> D-Scope8/2  "<i_dq>"
  DS-Bus8/3 -> D-Scope8/3  "<v_abc>"
  DS-Bus8/4 -> D-Scope8/4  "<i_abc>"
  DS-Bus8/5 -> D-Scope8/5  "<w>"
  DS-Bus8/6 -> D-Scope8/6  "<theta>"
  DS-Bus8/7 -> D-Scope8/7  "<pq>"
  SM_8th_AVRPSSGOV9/1 -> DS-Bus9/1
  DS-Bus9/1 -> D-Scope9/1  "<v_dq>"
  DS-Bus9/2 -> D-Scope9/2  "<i_dq>"
  DS-Bus9/3 -> D-Scope9/3  "<v_abc>"
  DS-Bus9/4 -> D-Scope9/4  "<i_abc>"
  DS-Bus9/5 -> D-Scope9/5  "<w>"
  DS-Bus9/6 -> D-Scope9/6  "<theta>"
  DS-Bus9/7 -> D-Scope9/7  "<pq>"
  SM_8th_AVRPSSGOV10/1 -> DS-Bus10/1
  DS-Bus10/1 -> D-Scope10/1  "<v_dq>"
  DS-Bus10/2 -> D-Scope10/2  "<i_dq>"
  DS-Bus10/3 -> D-Scope10/3  "<v_abc>"
  DS-Bus10/4 -> D-Scope10/4  "<i_abc>"
  DS-Bus10/5 -> D-Scope10/5  "<w>"
  DS-Bus10/6 -> D-Scope10/6  "<theta>"
  DS-Bus10/7 -> D-Scope10/7  "<pq>"
  SM_8th_AVRPSSGOV11/1 -> DS-Bus11/1
  DS-Bus11/1 -> D-Scope11/1  "<v_dq>"
  DS-Bus11/2 -> D-Scope11/2  "<i_dq>"
  DS-Bus11/3 -> D-Scope11/3  "<v_abc>"
  DS-Bus11/4 -> D-Scope11/4  "<i_abc>"
  DS-Bus11/5 -> D-Scope11/5  "<w>"
  DS-Bus11/6 -> D-Scope11/6  "<theta>"
  DS-Bus11/7 -> D-Scope11/7  "<pq>"
  SM_8th_AVRPSSGOV12/1 -> DS-Bus12/1
  DS-Bus12/1 -> D-Scope12/1  "<v_dq>"
  DS-Bus12/2 -> D-Scope12/2  "<i_dq>"
  DS-Bus12/3 -> D-Scope12/3  "<v_abc>"
  DS-Bus12/4 -> D-Scope12/4  "<i_abc>"
  DS-Bus12/5 -> D-Scope12/5  "<w>"
  DS-Bus12/6 -> D-Scope12/6  "<theta>"
  DS-Bus12/7 -> D-Scope12/7  "<pq>"
  SM_8th_GOV13/1 -> DS-Bus13/1
  DS-Bus13/1 -> D-Scope13/1  "<v_dq>"
  DS-Bus13/2 -> D-Scope13/2  "<i_dq>"
  DS-Bus13/3 -> D-Scope13/3  "<v_abc>"
  DS-Bus13/4 -> D-Scope13/4  "<i_abc>"
  DS-Bus13/5 -> D-Scope13/5  "<w>"
  DS-Bus13/6 -> D-Scope13/6  "<theta>"
  DS-Bus13/7 -> D-Scope13/7  "<pq>"
  SM_8th_GOV14/1 -> DS-Bus14/1
  DS-Bus14/1 -> D-Scope14/1  "<v_dq>"
  DS-Bus14/2 -> D-Scope14/2  "<i_dq>"
  DS-Bus14/3 -> D-Scope14/3  "<v_abc>"
  DS-Bus14/4 -> D-Scope14/4  "<i_abc>"
  DS-Bus14/5 -> D-Scope14/5  "<w>"
  DS-Bus14/6 -> D-Scope14/6  "<theta>"
  DS-Bus14/7 -> D-Scope14/7  "<pq>"
  SM_8th_GOV15/1 -> DS-Bus15/1
  DS-Bus15/1 -> D-Scope15/1  "<v_dq>"
  DS-Bus15/2 -> D-Scope15/2  "<i_dq>"
  DS-Bus15/3 -> D-Scope15/3  "<v_abc>"
  DS-Bus15/4 -> D-Scope15/4  "<i_abc>"
  DS-Bus15/5 -> D-Scope15/5  "<w>"
  DS-Bus15/6 -> D-Scope15/6  "<theta>"
  DS-Bus15/7 -> D-Scope15/7  "<pq>"
  SM_8th_AVRPSSGOV16/1 -> DS-Bus16/1
  DS-Bus16/1 -> D-Scope16/1  "<v_dq>"
  DS-Bus16/2 -> D-Scope16/2  "<i_dq>"
  DS-Bus16/3 -> D-Scope16/3  "<v_abc>"
  DS-Bus16/4 -> D-Scope16/4  "<i_abc>"
  DS-Bus16/5 -> D-Scope16/5  "<w>"
  DS-Bus16/6 -> D-Scope16/6  "<theta>"
  DS-Bus16/7 -> D-Scope16/7  "<pq>"
  VSI-PLL17/1 -> DS-Bus17/1
  DS-Bus17/1 -> D-Scope17/1  "<v_dq>"
  DS-Bus17/2 -> D-Scope17/2  "<i_dq>"
  DS-Bus17/3 -> D-Scope17/3  "<v_abc>"
  DS-Bus17/4 -> D-Scope17/4  "<i_abc>"
  DS-Bus17/5 -> D-Scope17/5  "<w>"
  DS-Bus17/6 -> D-Scope17/6  "<theta>"
  DS-Bus17/7 -> D-Scope17/7  "<pq>"
  VSI-PLL26/1 -> DS-Bus26/1
  DS-Bus26/1 -> D-Scope26/1  "<v_dq>"
  DS-Bus26/2 -> D-Scope26/2  "<i_dq>"
  DS-Bus26/3 -> D-Scope26/3  "<v_abc>"
  DS-Bus26/4 -> D-Scope26/4  "<i_abc>"
  DS-Bus26/5 -> D-Scope26/5  "<w>"
  DS-Bus26/6 -> D-Scope26/6  "<theta>"
  DS-Bus26/7 -> D-Scope26/7  "<pq>"
  VSI-PLL27/1 -> DS-Bus27/1
  DS-Bus27/1 -> D-Scope27/1  "<v_dq>"
  DS-Bus27/2 -> D-Scope27/2  "<i_dq>"
  DS-Bus27/3 -> D-Scope27/3  "<v_abc>"
  DS-Bus27/4 -> D-Scope27/4  "<i_abc>"
  DS-Bus27/5 -> D-Scope27/5  "<w>"
  DS-Bus27/6 -> D-Scope27/6  "<theta>"
  DS-Bus27/7 -> D-Scope27/7  "<pq>"
  VSI-PLL28/1 -> DS-Bus28/1
  DS-Bus28/1 -> D-Scope28/1  "<v_dq>"
  DS-Bus28/2 -> D-Scope28/2  "<i_dq>"
  DS-Bus28/3 -> D-Scope28/3  "<v_abc>"
  DS-Bus28/4 -> D-Scope28/4  "<i_abc>"
  DS-Bus28/5 -> D-Scope28/5  "<w>"
  DS-Bus28/6 -> D-Scope28/6  "<theta>"
  DS-Bus28/7 -> D-Scope28/7  "<pq>"
  VSI-PLL29/1 -> DS-Bus29/1
  DS-Bus29/1 -> D-Scope29/1  "<v_dq>"
  DS-Bus29/2 -> D-Scope29/2  "<i_dq>"
  DS-Bus29/3 -> D-Scope29/3  "<v_abc>"
  DS-Bus29/4 -> D-Scope29/4  "<i_abc>"
  DS-Bus29/5 -> D-Scope29/5  "<w>"
  DS-Bus29/6 -> D-Scope29/6  "<theta>"
  DS-Bus29/7 -> D-Scope29/7  "<pq>"
  VSI-PLL35/1 -> DS-Bus35/1
  DS-Bus35/1 -> D-Scope35/1  "<v_dq>"
  DS-Bus35/2 -> D-Scope35/2  "<i_dq>"
  DS-Bus35/3 -> D-Scope35/3  "<v_abc>"
  DS-Bus35/4 -> D-Scope35/4  "<i_abc>"
  DS-Bus35/5 -> D-Scope35/5  "<w>"
  DS-Bus35/6 -> D-Scope35/6  "<theta>"
  DS-Bus35/7 -> D-Scope35/7  "<pq>"
  VSI-PLL39/1 -> DS-Bus39/1
  DS-Bus39/1 -> D-Scope39/1  "<v_dq>"
  DS-Bus39/2 -> D-Scope39/2  "<i_dq>"
  DS-Bus39/3 -> D-Scope39/3  "<v_abc>"
  DS-Bus39/4 -> D-Scope39/4  "<i_abc>"
  DS-Bus39/5 -> D-Scope39/5  "<w>"
  DS-Bus39/6 -> D-Scope39/6  "<theta>"
  DS-Bus39/7 -> D-Scope39/7  "<pq>"
  VSI-PLL43/1 -> DS-Bus43/1
  DS-Bus43/1 -> D-Scope43/1  "<v_dq>"
  DS-Bus43/2 -> D-Scope43/2  "<i_dq>"
  DS-Bus43/3 -> D-Scope43/3  "<v_abc>"
  DS-Bus43/4 -> D-Scope43/4  "<i_abc>"
  DS-Bus43/5 -> D-Scope43/5  "<w>"
  DS-Bus43/6 -> D-Scope43/6  "<theta>"
  DS-Bus43/7 -> D-Scope43/7  "<pq>"
  VSI-PLL44/1 -> DS-Bus44/1
  DS-Bus44/1 -> D-Scope44/1  "<v_dq>"
  DS-Bus44/2 -> D-Scope44/2  "<i_dq>"
  DS-Bus44/3 -> D-Scope44/3  "<v_abc>"
  DS-Bus44/4 -> D-Scope44/4  "<i_abc>"
  DS-Bus44/5 -> D-Scope44/5  "<w>"
  DS-Bus44/6 -> D-Scope44/6  "<theta>"
  DS-Bus44/7 -> D-Scope44/7  "<pq>"
  VSI-PLL45/1 -> DS-Bus45/1
  DS-Bus45/1 -> D-Scope45/1  "<v_dq>"
  DS-Bus45/2 -> D-Scope45/2  "<i_dq>"
  DS-Bus45/3 -> D-Scope45/3  "<v_abc>"
  DS-Bus45/4 -> D-Scope45/4  "<i_abc>"
  DS-Bus45/5 -> D-Scope45/5  "<w>"
  DS-Bus45/6 -> D-Scope45/6  "<theta>"
  DS-Bus45/7 -> D-Scope45/7  "<pq>"
  VSI-PLL50/1 -> DS-Bus50/1
  DS-Bus50/1 -> D-Scope50/1  "<v_dq>"
  DS-Bus50/2 -> D-Scope50/2  "<i_dq>"
  DS-Bus50/3 -> D-Scope50/3  "<v_abc>"
  DS-Bus50/4 -> D-Scope50/4  "<i_abc>"
  DS-Bus50/5 -> D-Scope50/5  "<w>"
  DS-Bus50/6 -> D-Scope50/6  "<theta>"
  DS-Bus50/7 -> D-Scope50/7  "<pq>"
  VSI-PLL51/1 -> DS-Bus51/1
  DS-Bus51/1 -> D-Scope51/1  "<v_dq>"
  DS-Bus51/2 -> D-Scope51/2  "<i_dq>"
  DS-Bus51/3 -> D-Scope51/3  "<v_abc>"
  DS-Bus51/4 -> D-Scope51/4  "<i_abc>"
  DS-Bus51/5 -> D-Scope51/5  "<w>"
  DS-Bus51/6 -> D-Scope51/6  "<theta>"
  DS-Bus51/7 -> D-Scope51/7  "<pq>"
  VSI-PLL58/1 -> DS-Bus58/1
  DS-Bus58/1 -> D-Scope58/1  "<v_dq>"
  DS-Bus58/2 -> D-Scope58/2  "<i_dq>"
  DS-Bus58/3 -> D-Scope58/3  "<v_abc>"
  DS-Bus58/4 -> D-Scope58/4  "<i_abc>"
  DS-Bus58/5 -> D-Scope58/5  "<w>"
  DS-Bus58/6 -> D-Scope58/6  "<theta>"
  DS-Bus58/7 -> D-Scope58/7  "<pq>"
  VSI-PLL59/1 -> DS-Bus59/1
  DS-Bus59/1 -> D-Scope59/1  "<v_dq>"
  DS-Bus59/2 -> D-Scope59/2  "<i_dq>"
  DS-Bus59/3 -> D-Scope59/3  "<v_abc>"
  DS-Bus59/4 -> D-Scope59/4  "<i_abc>"
  DS-Bus59/5 -> D-Scope59/5  "<w>"
  DS-Bus59/6 -> D-Scope59/6  "<theta>"
  DS-Bus59/7 -> D-Scope59/7  "<pq>"
  connections:
  SM_8th_GOV1/LConn4 -- D-GND1/LConn1
  SM_8th_AVRPSSGOV2/LConn4 -- D-GND2/LConn1
  SM_8th_AVRPSSGOV3/LConn4 -- D-GND3/LConn1
  SM_8th_AVRPSSGOV4/LConn4 -- D-GND4/LConn1
  SM_8th_AVRPSSGOV5/LConn4 -- D-GND5/LConn1
  SM_8th_AVRPSSGOV6/LConn4 -- D-GND6/LConn1
  SM_8th_AVRPSSGOV7/LConn4 -- D-GND7/LConn1
  SM_8th_AVRPSSGOV8/LConn4 -- D-GND8/LConn1
  SM_8th_AVRPSSGOV9/LConn4 -- D-GND9/LConn1
  SM_8th_AVRPSSGOV10/LConn4 -- D-GND10/LConn1
  SM_8th_AVRPSSGOV11/LConn4 -- D-GND11/LConn1
  SM_8th_AVRPSSGOV12/LConn4 -- D-GND12/LConn1
  SM_8th_GOV13/LConn4 -- D-GND13/LConn1
  SM_8th_GOV14/LConn4 -- D-GND14/LConn1
  SM_8th_GOV15/LConn4 -- D-GND15/LConn1
  SM_8th_AVRPSSGOV16/LConn4 -- D-GND16/LConn1
  VSI-PLL17/LConn4 -- D-GND17/LConn1
  VSI-PLL26/LConn4 -- D-GND26/LConn1
  VSI-PLL27/LConn4 -- D-GND27/LConn1
  VSI-PLL28/LConn4 -- D-GND28/LConn1
  VSI-PLL29/LConn4 -- D-GND29/LConn1
  VSI-PLL35/LConn4 -- D-GND35/LConn1
  VSI-PLL39/LConn4 -- D-GND39/LConn1
  VSI-PLL43/LConn4 -- D-GND43/LConn1
  VSI-PLL44/LConn4 -- D-GND44/LConn1
  VSI-PLL45/LConn4 -- D-GND45/LConn1
  VSI-PLL50/LConn4 -- D-GND50/LConn1
  VSI-PLL51/LConn4 -- D-GND51/LConn1
  VSI-PLL58/LConn4 -- D-GND58/LConn1
  VSI-PLL59/LConn4 -- D-GND59/LConn1
  Branch1-1/RConn1 -- Branch1-1/RConn2 -- Branch1-1/RConn3 -- B-GND1/LConn1
  Branch2-2/RConn1 -- Branch2-2/RConn2 -- Branch2-2/RConn3 -- B-GND3/LConn1
  Branch3-3/RConn1 -- Branch3-3/RConn2 -- Branch3-3/RConn3 -- B-GND5/LConn1
  Branch4-4/RConn1 -- Branch4-4/RConn2 -- Branch4-4/RConn3 -- B-GND7/LConn1
  Branch5-5/RConn1 -- Branch5-5/RConn2 -- Branch5-5/RConn3 -- B-GND9/LConn1
  Branch6-6/RConn1 -- Branch6-6/RConn2 -- Branch6-6/RConn3 -- B-GND11/LConn1
  Branch7-7/RConn1 -- Branch7-7/RConn2 -- Branch7-7/RConn3 -- B-GND13/LConn1
  Branch8-8/RConn1 -- Branch8-8/RConn2 -- Branch8-8/RConn3 -- B-GND15/LConn1
  Branch9-9/RConn1 -- Branch9-9/RConn2 -- Branch9-9/RConn3 -- B-GND17/LConn1
  Branch10-10/RConn1 -- Branch10-10/RConn2 -- Branch10-10/RConn3 -- B-GND19/LConn1
  Branch11-11/RConn1 -- Branch11-11/RConn2 -- Branch11-11/RConn3 -- B-GND21/LConn1
  Branch12-12/RConn1 -- Branch12-12/RConn2 -- Branch12-12/RConn3 -- B-GND23/LConn1
  Branch13-13/RConn1 -- Branch13-13/RConn2 -- Branch13-13/RConn3 -- B-GND25/LConn1
  Branch14-14/RConn1 -- Branch14-14/RConn2 -- Branch14-14/RConn3 -- B-GND27/LConn1
  Branch15-15/RConn1 -- Branch15-15/RConn2 -- Branch15-15/RConn3 -- B-GND29/LConn1
  Branch16-16/RConn1 -- Branch16-16/RConn2 -- Branch16-16/RConn3 -- B-GND31/LConn1
  Branch17-17/RConn1 -- Branch17-17/RConn2 -- Branch17-17/RConn3 -- B-GND33/LConn1
  Branch18-18/RConn1 -- Branch18-18/RConn2 -- Branch18-18/RConn3 -- B-GND36/LConn1
  Branch19-19/RConn1 -- Branch19-19/RConn2 -- Branch19-19/RConn3 -- B-GND40/LConn1
  Branch20-20/RConn1 -- Branch20-20/RConn2 -- Branch20-20/RConn3 -- B-GND43/LConn1
  Branch21-21/RConn1 -- Branch21-21/RConn2 -- Branch21-21/RConn3 -- B-GND44/LConn1
  Branch22-22/RConn1 -- Branch22-22/RConn2 -- Branch22-22/RConn3 -- B-GND47/LConn1
  Branch23-23/RConn1 -- Branch23-23/RConn2 -- Branch23-23/RConn3 -- B-GND49/LConn1
  Branch24-24/RConn1 -- Branch24-24/RConn2 -- Branch24-24/RConn3 -- B-GND51/LConn1
  Branch25-25/RConn1 -- Branch25-25/RConn2 -- Branch25-25/RConn3 -- B-GND53/LConn1
  Branch26-26/RConn1 -- Branch26-26/RConn2 -- Branch26-26/RConn3 -- B-GND56/LConn1
  Branch27-27/RConn1 -- Branch27-27/RConn2 -- Branch27-27/RConn3 -- B-GND60/LConn1
  Branch28-28/RConn1 -- Branch28-28/RConn2 -- Branch28-28/RConn3 -- B-GND63/LConn1
  Branch29-29/RConn1 -- Branch29-29/RConn2 -- Branch29-29/RConn3 -- B-GND65/LConn1
  Branch30-30/RConn1 -- Branch30-30/RConn2 -- Branch30-30/RConn3 -- B-GND66/LConn1
  Branch31-31/RConn1 -- Branch31-31/RConn2 -- Branch31-31/RConn3 -- B-GND71/LConn1
  Branch32-32/RConn1 -- Branch32-32/RConn2 -- Branch32-32/RConn3 -- B-GND74/LConn1
  Branch33-33/RConn1 -- Branch33-33/RConn2 -- Branch33-33/RConn3 -- B-GND76/LConn1
  Branch34-34/RConn1 -- Branch34-34/RConn2 -- Branch34-34/RConn3 -- B-GND79/LConn1
  Branch35-35/RConn1 -- Branch35-35/RConn2 -- Branch35-35/RConn3 -- B-GND82/LConn1
  Branch36-36/RConn1 -- Branch36-36/RConn2 -- Branch36-36/RConn3 -- B-GND84/LConn1
  Branch37-37/RConn1 -- Branch37-37/RConn2 -- Branch37-37/RConn3 -- B-GND86/LConn1
  Branch38-38/RConn1 -- Branch38-38/RConn2 -- Branch38-38/RConn3 -- B-GND89/LConn1
  Branch39-39/RConn1 -- Branch39-39/RConn2 -- Branch39-39/RConn3 -- B-GND91/LConn1
  Branch40-40/RConn1 -- Branch40-40/RConn2 -- Branch40-40/RConn3 -- B-GND94/LConn1
  Branch41-41/RConn1 -- Branch41-41/RConn2 -- Branch41-41/RConn3 -- B-GND97/LConn1
  Branch42-42/RConn1 -- Branch42-42/RConn2 -- Branch42-42/RConn3 -- B-GND99/LConn1
  Branch43-43/RConn1 -- Branch43-43/RConn2 -- Branch43-43/RConn3 -- B-GND100/LConn1
  Branch44-44/RConn1 -- Branch44-44/RConn2 -- Branch44-44/RConn3 -- B-GND102/LConn1
  Branch45-45/RConn1 -- Branch45-45/RConn2 -- Branch45-45/RConn3 -- B-GND104/LConn1
  Branch46-46/RConn1 -- Branch46-46/RConn2 -- Branch46-46/RConn3 -- B-GND106/LConn1
  Branch47-47/RConn1 -- Branch47-47/RConn2 -- Branch47-47/RConn3 -- B-GND108/LConn1
  Branch48-48/RConn1 -- Branch48-48/RConn2 -- Branch48-48/RConn3 -- B-GND111/LConn1
  Branch49-49/RConn1 -- Branch49-49/RConn2 -- Branch49-49/RConn3 -- B-GND112/LConn1
  Branch50-50/RConn1 -- Branch50-50/RConn2 -- Branch50-50/RConn3 -- B-GND113/LConn1
  Branch51-51/RConn1 -- Branch51-51/RConn2 -- Branch51-51/RConn3 -- B-GND115/LConn1
  Branch52-52/RConn1 -- Branch52-52/RConn2 -- Branch52-52/RConn3 -- B-GND116/LConn1
  Branch53-53/RConn1 -- Branch53-53/RConn2 -- Branch53-53/RConn3 -- B-GND118/LConn1
  Branch54-54/RConn1 -- Branch54-54/RConn2 -- Branch54-54/RConn3 -- B-GND120/LConn1
  Branch55-55/RConn1 -- Branch55-55/RConn2 -- Branch55-55/RConn3 -- B-GND122/LConn1
  Branch56-56/RConn1 -- Branch56-56/RConn2 -- Branch56-56/RConn3 -- B-GND124/LConn1
  Branch57-57/RConn1 -- Branch57-57/RConn2 -- Branch57-57/RConn3 -- B-GND127/LConn1
  Branch58-58/RConn1 -- Branch58-58/RConn2 -- Branch58-58/RConn3 -- B-GND130/LConn1
  Branch59-59/RConn1 -- Branch59-59/RConn2 -- Branch59-59/RConn3 -- B-GND133/LConn1
  Branch60-60/RConn1 -- Branch60-60/RConn2 -- Branch60-60/RConn3 -- B-GND135/LConn1
  Branch61-61/RConn1 -- Branch61-61/RConn2 -- Branch61-61/RConn3 -- B-GND137/LConn1
  Branch62-62/RConn1 -- Branch62-62/RConn2 -- Branch62-62/RConn3 -- B-GND138/LConn1
  Branch63-63/RConn1 -- Branch63-63/RConn2 -- Branch63-63/RConn3 -- B-GND141/LConn1
  Branch64-64/RConn1 -- Branch64-64/RConn2 -- Branch64-64/RConn3 -- B-GND143/LConn1
  Branch65-65/RConn1 -- Branch65-65/RConn2 -- Branch65-65/RConn3 -- B-GND145/LConn1
  Branch66-66/RConn1 -- Branch66-66/RConn2 -- Branch66-66/RConn3 -- B-GND147/LConn1
  Branch67-67/RConn1 -- Branch67-67/RConn2 -- Branch67-67/RConn3 -- B-GND149/LConn1
  Branch68-68/RConn1 -- Branch68-68/RConn2 -- Branch68-68/RConn3 -- B-GND151/LConn1
  Branch1-18/RConn1 -- Bus18/RConn1 -- Branch18-18/LConn1 -- Branch18-50/LConn1 -- Branch18-49/LConn1 -- Branch18-42/LConn1
  Branch1-18/RConn2 -- Bus18/RConn2 -- Branch18-18/LConn2 -- Branch18-50/LConn2 -- Branch18-49/LConn2 -- Branch18-42/LConn2
  Branch1-18/RConn3 -- Bus18/RConn3 -- Branch18-18/LConn3 -- Branch18-50/LConn3 -- Branch18-49/LConn3 -- Branch18-42/LConn3
  Branch1-18/LConn1 -- Bus1/RConn1 -- Branch1-1/LConn1
  Branch1-18/LConn2 -- Bus1/RConn2 -- Branch1-1/LConn2
  Branch1-18/LConn3 -- Bus1/RConn3 -- Branch1-1/LConn3
  Branch2-58/RConn1 -- Bus58/RConn1 -- Branch58-58/LConn1 -- Branch58-63/LConn1 -- Branch58-59/LConn1 -- Branch57-58/RConn1
  Branch2-58/RConn2 -- Bus58/RConn2 -- Branch58-58/LConn2 -- Branch58-63/LConn2 -- Branch58-59/LConn2 -- Branch57-58/RConn2
  Branch2-58/RConn3 -- Bus58/RConn3 -- Branch58-58/LConn3 -- Branch58-63/LConn3 -- Branch58-59/LConn3 -- Branch57-58/RConn3
  Transformer2-58/RConn1 -- Branch2-58/LConn1
  Transformer2-58/RConn2 -- Branch2-58/LConn2
  Transformer2-58/RConn3 -- Branch2-58/LConn3
  Transformer2-58/LConn1 -- Bus2/RConn1 -- Branch2-2/LConn1
  Transformer2-58/LConn2 -- Bus2/RConn2 -- Branch2-2/LConn2
  Transformer2-58/LConn3 -- Bus2/RConn3 -- Branch2-2/LConn3
  Branch3-62/RConn1 -- Bus62/RConn1 -- Branch62-62/LConn1 -- Branch62-65/LConn1 -- Branch62-63/LConn1
  Branch3-62/RConn2 -- Bus62/RConn2 -- Branch62-62/LConn2 -- Branch62-65/LConn2 -- Branch62-63/LConn2
  Branch3-62/RConn3 -- Bus62/RConn3 -- Branch62-62/LConn3 -- Branch62-65/LConn3 -- Branch62-63/LConn3
  Transformer3-62/RConn1 -- Branch3-62/LConn1
  Transformer3-62/RConn2 -- Branch3-62/LConn2
  Transformer3-62/RConn3 -- Branch3-62/LConn3
  Transformer3-62/LConn1 -- Bus3/RConn1 -- Branch3-3/LConn1
  Transformer3-62/LConn2 -- Bus3/RConn2 -- Branch3-3/LConn2
  Transformer3-62/LConn3 -- Bus3/RConn3 -- Branch3-3/LConn3
  Branch4-19/RConn1 -- Bus19/RConn1 -- Branch19-19/LConn1 -- Branch19-68/LConn1 -- Transformer19-20/LConn1
  Branch4-19/RConn2 -- Bus19/RConn2 -- Branch19-19/LConn2 -- Branch19-68/LConn2 -- Transformer19-20/LConn2
  Branch4-19/RConn3 -- Bus19/RConn3 -- Branch19-19/LConn3 -- Branch19-68/LConn3 -- Transformer19-20/LConn3
  Transformer4-19/RConn1 -- Branch4-19/LConn1
  Transformer4-19/RConn2 -- Branch4-19/LConn2
  Transformer4-19/RConn3 -- Branch4-19/LConn3
  Transformer4-19/LConn1 -- Bus4/RConn1 -- Branch4-4/LConn1
  Transformer4-19/LConn2 -- Bus4/RConn2 -- Branch4-4/LConn2
  Transformer4-19/LConn3 -- Bus4/RConn3 -- Branch4-4/LConn3
  Branch5-20/RConn1 -- Bus20/RConn1 -- Branch20-20/LConn1 -- Branch19-20/RConn1
  Branch5-20/RConn2 -- Bus20/RConn2 -- Branch20-20/LConn2 -- Branch19-20/RConn2
  Branch5-20/RConn3 -- Bus20/RConn3 -- Branch20-20/LConn3 -- Branch19-20/RConn3
  Transformer5-20/RConn1 -- Branch5-20/LConn1
  Transformer5-20/RConn2 -- Branch5-20/LConn2
  Transformer5-20/RConn3 -- Branch5-20/LConn3
  Transformer5-20/LConn1 -- Bus5/RConn1 -- Branch5-5/LConn1
  Transformer5-20/LConn2 -- Bus5/RConn2 -- Branch5-5/LConn2
  Transformer5-20/LConn3 -- Bus5/RConn3 -- Branch5-5/LConn3
  Branch6-22/RConn1 -- Bus22/RConn1 -- Branch22-22/LConn1 -- Branch22-23/LConn1 -- Branch21-22/RConn1
  Branch6-22/RConn2 -- Bus22/RConn2 -- Branch22-22/LConn2 -- Branch22-23/LConn2 -- Branch21-22/RConn2
  Branch6-22/RConn3 -- Bus22/RConn3 -- Branch22-22/LConn3 -- Branch22-23/LConn3 -- Branch21-22/RConn3
  Transformer6-22/RConn1 -- Branch6-22/LConn1
  Transformer6-22/RConn2 -- Branch6-22/LConn2
  Transformer6-22/RConn3 -- Branch6-22/LConn3
  Transformer6-22/LConn1 -- Bus6/RConn1 -- Branch6-6/LConn1
  Transformer6-22/LConn2 -- Bus6/RConn2 -- Branch6-6/LConn2
  Transformer6-22/LConn3 -- Bus6/RConn3 -- Branch6-6/LConn3
  Branch7-23/RConn1 -- Bus23/RConn1 -- Branch23-23/LConn1 -- Branch23-24/LConn1 -- Branch22-23/RConn1
  Branch7-23/RConn2 -- Bus23/RConn2 -- Branch23-23/LConn2 -- Branch23-24/LConn2 -- Branch22-23/RConn2
  Branch7-23/RConn3 -- Bus23/RConn3 -- Branch23-23/LConn3 -- Branch23-24/LConn3 -- Branch22-23/RConn3
  Branch7-23/LConn1 -- Bus7/RConn1 -- Branch7-7/LConn1
  Branch7-23/LConn2 -- Bus7/RConn2 -- Branch7-7/LConn2
  Branch7-23/LConn3 -- Bus7/RConn3 -- Branch7-7/LConn3
  Branch8-25/RConn1 -- Bus25/RConn1 -- Branch25-25/LConn1 -- Branch25-54/LConn1 -- Branch25-26/LConn1
  Branch8-25/RConn2 -- Bus25/RConn2 -- Branch25-25/LConn2 -- Branch25-54/LConn2 -- Branch25-26/LConn2
  Branch8-25/RConn3 -- Bus25/RConn3 -- Branch25-25/LConn3 -- Branch25-54/LConn3 -- Branch25-26/LConn3
  Transformer8-25/RConn1 -- Branch8-25/LConn1
  Transformer8-25/RConn2 -- Branch8-25/LConn2
  Transformer8-25/RConn3 -- Branch8-25/LConn3
  Transformer8-25/LConn1 -- Bus8/RConn1 -- Branch8-8/LConn1
  Transformer8-25/LConn2 -- Bus8/RConn2 -- Branch8-8/LConn2
  Transformer8-25/LConn3 -- Bus8/RConn3 -- Branch8-8/LConn3
  Branch9-29/RConn1 -- Three-Phase Breaker2/LConn1 -- Branch28-29/RConn1 -- Branch26-29/RConn1 -- Branch29-29/LConn1 -- Bus29/RConn1
  Branch9-29/RConn2 -- Bus29/RConn2 -- Branch29-29/LConn2 -- Branch28-29/RConn2 -- Three-Phase Breaker2/LConn2 -- Branch26-29/RConn2
  Branch9-29/RConn3 -- Bus29/RConn3 -- Branch29-29/LConn3 -- Three-Phase Breaker2/LConn3 -- Branch28-29/RConn3 -- Branch26-29/RConn3
  Transformer9-29/RConn1 -- Branch9-29/LConn1
  Transformer9-29/RConn2 -- Branch9-29/LConn2
  Transformer9-29/RConn3 -- Branch9-29/LConn3
  Transformer9-29/LConn1 -- Bus9/RConn1 -- Branch9-9/LConn1
  Transformer9-29/LConn2 -- Bus9/RConn2 -- Branch9-9/LConn2
  Transformer9-29/LConn3 -- Bus9/RConn3 -- Branch9-9/LConn3
  Branch10-31/RConn1 -- Bus31/RConn1 -- Branch31-31/LConn1 -- Branch31-53/LConn1 -- Branch31-38/LConn1 -- Branch30-31/RConn1
  Branch10-31/RConn2 -- Bus31/RConn2 -- Branch31-31/LConn2 -- Branch31-53/LConn2 -- Branch31-38/LConn2 -- Branch30-31/RConn2
  Branch10-31/RConn3 -- Bus31/RConn3 -- Branch31-31/LConn3 -- Branch31-53/LConn3 -- Branch31-38/LConn3 -- Branch30-31/RConn3
  Transformer10-31/RConn1 -- Branch10-31/LConn1
  Transformer10-31/RConn2 -- Branch10-31/LConn2
  Transformer10-31/RConn3 -- Branch10-31/LConn3
  Transformer10-31/LConn1 -- Bus10/RConn1 -- Branch10-10/LConn1
  Transformer10-31/LConn2 -- Bus10/RConn2 -- Branch10-10/LConn2
  Transformer10-31/LConn3 -- Bus10/RConn3 -- Branch10-10/LConn3
  Branch11-32/RConn1 -- Bus32/RConn1 -- Branch32-32/LConn1 -- Branch32-33/LConn1 -- Branch30-32/RConn1
  Branch11-32/RConn2 -- Bus32/RConn2 -- Branch32-32/LConn2 -- Branch32-33/LConn2 -- Branch30-32/RConn2
  Branch11-32/RConn3 -- Bus32/RConn3 -- Branch32-32/LConn3 -- Branch32-33/LConn3 -- Branch30-32/RConn3
  Transformer11-32/RConn1 -- Branch11-32/LConn1
  Transformer11-32/RConn2 -- Branch11-32/LConn2
  Transformer11-32/RConn3 -- Branch11-32/LConn3
  Transformer11-32/LConn1 -- Bus11/RConn1 -- Branch11-11/LConn1
  Transformer11-32/LConn2 -- Bus11/RConn2 -- Branch11-11/LConn2
  Transformer11-32/LConn3 -- Bus11/RConn3 -- Branch11-11/LConn3
  Branch12-36/RConn1 -- Bus36/RConn1 -- Branch36-36/LConn1 -- Branch36-61/LConn1 -- Branch34-36/RConn1 -- Branch17-36/RConn1
  Branch12-36/RConn2 -- Bus36/RConn2 -- Branch36-36/LConn2 -- Branch36-61/LConn2 -- Branch34-36/RConn2 -- Branch17-36/RConn2
  Branch12-36/RConn3 -- Bus36/RConn3 -- Branch36-36/LConn3 -- Branch36-61/LConn3 -- Branch34-36/RConn3 -- Branch17-36/RConn3
  Transformer12-36/RConn1 -- Branch12-36/LConn1
  Transformer12-36/RConn2 -- Branch12-36/LConn2
  Transformer12-36/RConn3 -- Branch12-36/LConn3
  Transformer12-36/LConn1 -- Bus12/RConn1 -- Branch12-12/LConn1
  Transformer12-36/LConn2 -- Bus12/RConn2 -- Branch12-12/LConn2
  Transformer12-36/LConn3 -- Bus12/RConn3 -- Branch12-12/LConn3
  Branch13-17/RConn1 -- Bus17/RConn1 -- Branch17-17/LConn1 -- Branch17-43/LConn1 -- Branch17-36/LConn1
  Branch13-17/RConn2 -- Bus17/RConn2 -- Branch17-17/LConn2 -- Branch17-43/LConn2 -- Branch17-36/LConn2
  Branch13-17/RConn3 -- Bus17/RConn3 -- Branch17-17/LConn3 -- Branch17-43/LConn3 -- Branch17-36/LConn3
  Transformer13-17/RConn1 -- Branch13-17/LConn1
  Transformer13-17/RConn2 -- Branch13-17/LConn2
  Transformer13-17/RConn3 -- Branch13-17/LConn3
  Transformer13-17/LConn1 -- Bus13/RConn1 -- Branch13-13/LConn1
  Transformer13-17/LConn2 -- Bus13/RConn2 -- Branch13-13/LConn2
  Transformer13-17/LConn3 -- Bus13/RConn3 -- Branch13-13/LConn3
  Branch14-41/RConn1 -- Bus41/RConn1 -- Branch41-41/LConn1 -- Branch41-42/LConn1 -- Branch40-41/RConn1
  Branch14-41/RConn2 -- Bus41/RConn2 -- Branch41-41/LConn2 -- Branch41-42/LConn2 -- Branch40-41/RConn2
  Branch14-41/RConn3 -- Bus41/RConn3 -- Branch41-41/LConn3 -- Branch41-42/LConn3 -- Branch40-41/RConn3
  Branch14-41/LConn1 -- Bus14/RConn1 -- Branch14-14/LConn1
  Branch14-41/LConn2 -- Bus14/RConn2 -- Branch14-14/LConn2
  Branch14-41/LConn3 -- Bus14/RConn3 -- Branch14-14/LConn3
  Branch15-42/RConn1 -- Bus42/RConn1 -- Branch42-42/LConn1 -- Branch41-42/RConn1 -- Branch18-42/RConn1
  Branch15-42/RConn2 -- Bus42/RConn2 -- Branch42-42/LConn2 -- Branch41-42/RConn2 -- Branch18-42/RConn2
  Branch15-42/RConn3 -- Bus42/RConn3 -- Branch42-42/LConn3 -- Branch41-42/RConn3 -- Branch18-42/RConn3
  Branch15-42/LConn1 -- Bus15/RConn1 -- Branch15-15/LConn1
  Branch15-42/LConn2 -- Bus15/RConn2 -- Branch15-15/LConn2
  Branch15-42/LConn3 -- Bus15/RConn3 -- Branch15-15/LConn3
  Branch16-54/RConn1 -- Bus54/RConn1 -- Branch54-54/LConn1 -- Branch54-55/LConn1 -- Branch53-54/RConn1 -- Branch25-54/RConn1
  Branch16-54/RConn2 -- Bus54/RConn2 -- Branch54-54/LConn2 -- Branch54-55/LConn2 -- Branch53-54/RConn2 -- Branch25-54/RConn2
  Branch16-54/RConn3 -- Bus54/RConn3 -- Branch54-54/LConn3 -- Branch54-55/LConn3 -- Branch53-54/RConn3 -- Branch25-54/RConn3
  Transformer16-54/RConn1 -- Branch16-54/LConn1
  Transformer16-54/RConn2 -- Branch16-54/LConn2
  Transformer16-54/RConn3 -- Branch16-54/LConn3
  Transformer16-54/LConn1 -- Bus16/RConn1 -- Branch16-16/LConn1
  Transformer16-54/LConn2 -- Bus16/RConn2 -- Branch16-16/LConn2
  Transformer16-54/LConn3 -- Bus16/RConn3 -- Branch16-16/LConn3
  Branch17-43/RConn1 -- Bus43/RConn1 -- Branch43-43/LConn1 -- Branch43-44/LConn1
  Branch17-43/RConn2 -- Bus43/RConn2 -- Branch43-43/LConn2 -- Branch43-44/LConn2
  Branch17-43/RConn3 -- Bus43/RConn3 -- Branch43-43/LConn3 -- Branch43-44/LConn3
  Branch18-49/RConn1 -- Bus49/RConn1 -- Branch49-49/LConn1 -- Branch46-49/RConn1
  Branch18-49/RConn2 -- Bus49/RConn2 -- Branch49-49/LConn2 -- Branch46-49/RConn2
  Branch18-49/RConn3 -- Bus49/RConn3 -- Branch49-49/LConn3 -- Branch46-49/RConn3
  Branch18-50/RConn1 -- Bus50/RConn1 -- Branch50-50/LConn1 -- Branch50-51/LConn1
  Branch18-50/RConn2 -- Bus50/RConn2 -- Branch50-50/LConn2 -- Branch50-51/LConn2
  Branch18-50/RConn3 -- Bus50/RConn3 -- Branch50-50/LConn3 -- Branch50-51/LConn3
  Transformer19-20/RConn1 -- Branch19-20/LConn1
  Transformer19-20/RConn2 -- Branch19-20/LConn2
  Transformer19-20/RConn3 -- Branch19-20/LConn3
  Branch19-68/RConn1 -- Bus68/RConn1 -- Branch68-68/LConn1 -- Branch67-68/RConn1 -- Branch37-68/RConn1 -- Branch24-68/RConn1 -- Branch21-68/RConn1
  Branch19-68/RConn2 -- Bus68/RConn2 -- Branch68-68/LConn2 -- Branch67-68/RConn2 -- Branch37-68/RConn2 -- Branch24-68/RConn2 -- Branch21-68/RConn2
  Branch19-68/RConn3 -- Bus68/RConn3 -- Branch68-68/LConn3 -- Branch67-68/RConn3 -- Branch37-68/RConn3 -- Branch24-68/RConn3 -- Branch21-68/RConn3
  Branch21-22/LConn1 -- Bus21/RConn1 -- Branch21-21/LConn1 -- Branch21-68/LConn1
  Branch21-22/LConn2 -- Bus21/RConn2 -- Branch21-21/LConn2 -- Branch21-68/LConn2
  Branch21-22/LConn3 -- Bus21/RConn3 -- Branch21-21/LConn3 -- Branch21-68/LConn3
  Branch23-24/RConn1 -- Bus24/RConn1 -- Branch24-24/LConn1 -- Branch24-68/LConn1
  Branch23-24/RConn2 -- Bus24/RConn2 -- Branch24-24/LConn2 -- Branch24-68/LConn2
  Branch23-24/RConn3 -- Bus24/RConn3 -- Branch24-24/LConn3 -- Branch24-68/LConn3
  Branch25-26/RConn1 -- Bus26/RConn1 -- Branch26-26/LConn1 -- Three-Phase Breaker/LConn1 -- Branch26-29/LConn1 -- Branch26-28/LConn1 -- Branch26-27/LConn1
  Branch25-26/RConn2 -- Bus26/RConn2 -- Branch26-26/LConn2 -- Three-Phase Breaker/LConn2 -- Branch26-29/LConn2 -- Branch26-28/LConn2 -- Branch26-27/LConn2
  Branch25-26/RConn3 -- Bus26/RConn3 -- Branch26-26/LConn3 -- Branch26-29/LConn3 -- Branch26-28/LConn3 -- Branch26-27/LConn3 -- Three-Phase Breaker/LConn3
  Branch26-27/RConn1 -- Bus27/RConn1 -- Branch27-27/LConn1 -- Branch27-53/LConn1 -- Branch27-37/LConn1
  Branch26-27/RConn2 -- Bus27/RConn2 -- Branch27-27/LConn2 -- Branch27-53/LConn2 -- Branch27-37/LConn2
  Branch26-27/RConn3 -- Bus27/RConn3 -- Branch27-27/LConn3 -- Branch27-53/LConn3 -- Branch27-37/LConn3
  Branch26-28/RConn1 -- Bus28/RConn1 -- Branch28-28/LConn1 -- Three-Phase Breaker1/LConn1 -- Branch28-29/LConn1
  Branch26-28/RConn2 -- Bus28/RConn2 -- Branch28-28/LConn2 -- Branch28-29/LConn2 -- Three-Phase Breaker1/LConn2
  Branch26-28/RConn3 -- Bus28/RConn3 -- Branch28-28/LConn3 -- Branch28-29/LConn3 -- Three-Phase Breaker1/LConn3
  Branch27-37/RConn1 -- Bus37/RConn1 -- Branch37-37/LConn1 -- Branch37-68/LConn1 -- Branch37-52/LConn1
  Branch27-37/RConn2 -- Bus37/RConn2 -- Branch37-37/LConn2 -- Branch37-68/LConn2 -- Branch37-52/LConn2
  Branch27-37/RConn3 -- Bus37/RConn3 -- Branch37-37/LConn3 -- Branch37-68/LConn3 -- Branch37-52/LConn3
  Branch27-53/RConn1 -- Bus53/RConn1 -- Branch53-53/LConn1 -- Branch53-54/LConn1 -- Branch47-53/RConn1 -- Branch31-53/RConn1 -- Branch30-53/RConn1
  Branch27-53/RConn2 -- Bus53/RConn2 -- Branch53-53/LConn2 -- Branch53-54/LConn2 -- Branch47-53/RConn2 -- Branch31-53/RConn2 -- Branch30-53/RConn2
  Branch27-53/RConn3 -- Bus53/RConn3 -- Branch53-53/LConn3 -- Branch53-54/LConn3 -- Branch47-53/RConn3 -- Branch31-53/RConn3 -- Branch30-53/RConn3
  Branch30-31/LConn1 -- Bus30/RConn1 -- Branch30-30/LConn1 -- Branch30-61/LConn1 -- Branch30-53/LConn1 -- Branch30-32/LConn1
  Branch30-31/LConn2 -- Bus30/RConn2 -- Branch30-30/LConn2 -- Branch30-61/LConn2 -- Branch30-53/LConn2 -- Branch30-32/LConn2
  Branch30-31/LConn3 -- Bus30/RConn3 -- Branch30-30/LConn3 -- Branch30-61/LConn3 -- Branch30-53/LConn3 -- Branch30-32/LConn3
  Branch30-61/RConn1 -- Bus61/RConn1 -- Branch61-61/LConn1 -- Branch60-61/RConn1 -- Branch36-61/RConn1
  Branch30-61/RConn2 -- Bus61/RConn2 -- Branch61-61/LConn2 -- Branch60-61/RConn2 -- Branch36-61/RConn2
  Branch30-61/RConn3 -- Bus61/RConn3 -- Branch61-61/LConn3 -- Branch60-61/RConn3 -- Branch36-61/RConn3
  Branch31-38/RConn1 -- Bus38/RConn1 -- Branch38-38/LConn1 -- Branch38-46/LConn1 -- Branch33-38/RConn1
  Branch31-38/RConn2 -- Bus38/RConn2 -- Branch38-38/LConn2 -- Branch38-46/LConn2 -- Branch33-38/RConn2
  Branch31-38/RConn3 -- Bus38/RConn3 -- Branch38-38/LConn3 -- Branch38-46/LConn3 -- Branch33-38/RConn3
  Branch32-33/RConn1 -- Bus33/RConn1 -- Branch33-33/LConn1 -- Branch33-38/LConn1 -- Branch33-34/LConn1
  Branch32-33/RConn2 -- Bus33/RConn2 -- Branch33-33/LConn2 -- Branch33-38/LConn2 -- Branch33-34/LConn2
  Branch32-33/RConn3 -- Bus33/RConn3 -- Branch33-33/LConn3 -- Branch33-38/LConn3 -- Branch33-34/LConn3
  Branch33-34/RConn1 -- Bus34/RConn1 -- Branch34-34/LConn1 -- Branch34-36/LConn1 -- Transformer34-35/LConn1
  Branch33-34/RConn2 -- Bus34/RConn2 -- Branch34-34/LConn2 -- Branch34-36/LConn2 -- Transformer34-35/LConn2
  Branch33-34/RConn3 -- Bus34/RConn3 -- Branch34-34/LConn3 -- Branch34-36/LConn3 -- Transformer34-35/LConn3
  Branch34-35/RConn1 -- Bus35/RConn1 -- Branch35-35/LConn1 -- Branch35-45/LConn1
  Branch34-35/RConn2 -- Bus35/RConn2 -- Branch35-35/LConn2 -- Branch35-45/LConn2
  Branch34-35/RConn3 -- Bus35/RConn3 -- Branch35-35/LConn3 -- Branch35-45/LConn3
  Transformer34-35/RConn1 -- Branch34-35/LConn1
  Transformer34-35/RConn2 -- Branch34-35/LConn2
  Transformer34-35/RConn3 -- Branch34-35/LConn3
  Branch35-45/RConn1 -- Bus45/RConn1 -- Branch45-45/LConn1 -- Branch45-51/LConn1 -- Branch44-45/RConn1 -- Branch39-45/RConn1
  Branch35-45/RConn2 -- Bus45/RConn2 -- Branch45-45/LConn2 -- Branch45-51/LConn2 -- Branch44-45/RConn2 -- Branch39-45/RConn2
  Branch35-45/RConn3 -- Bus45/RConn3 -- Branch45-45/LConn3 -- Branch45-51/LConn3 -- Branch44-45/RConn3 -- Branch39-45/RConn3
  Branch37-52/RConn1 -- Bus52/RConn1 -- Branch52-52/LConn1 -- Branch52-55/LConn1
  Branch37-52/RConn2 -- Bus52/RConn2 -- Branch52-52/LConn2 -- Branch52-55/LConn2
  Branch37-52/RConn3 -- Bus52/RConn3 -- Branch52-52/LConn3 -- Branch52-55/LConn3
  Branch38-46/RConn1 -- Bus46/RConn1 -- Branch46-46/LConn1 -- Branch46-49/LConn1
  Branch38-46/RConn2 -- Bus46/RConn2 -- Branch46-46/LConn2 -- Branch46-49/LConn2
  Branch38-46/RConn3 -- Bus46/RConn3 -- Branch46-46/LConn3 -- Branch46-49/LConn3
  Branch39-44/RConn1 -- Bus44/RConn1 -- Branch44-44/LConn1 -- Branch44-45/LConn1 -- Branch43-44/RConn1
  Branch39-44/RConn2 -- Bus44/RConn2 -- Branch44-44/LConn2 -- Branch44-45/LConn2 -- Branch43-44/RConn2
  Branch39-44/RConn3 -- Bus44/RConn3 -- Branch44-44/LConn3 -- Branch44-45/LConn3 -- Branch43-44/RConn3
  Branch39-44/LConn1 -- Bus39/RConn1 -- Branch39-39/LConn1 -- Branch39-45/LConn1
  Branch39-44/LConn2 -- Bus39/RConn2 -- Branch39-39/LConn2 -- Branch39-45/LConn2
  Branch39-44/LConn3 -- Bus39/RConn3 -- Branch39-39/LConn3 -- Branch39-45/LConn3
  Branch40-41/LConn1 -- Bus40/RConn1 -- Branch40-40/LConn1 -- Branch40-48/LConn1
  Branch40-41/LConn2 -- Bus40/RConn2 -- Branch40-40/LConn2 -- Branch40-48/LConn2
  Branch40-41/LConn3 -- Bus40/RConn3 -- Branch40-40/LConn3 -- Branch40-48/LConn3
  Branch40-48/RConn1 -- Bus48/RConn1 -- Branch48-48/LConn1 -- Branch47-48/RConn1
  Branch40-48/RConn2 -- Bus48/RConn2 -- Branch48-48/LConn2 -- Branch47-48/RConn2
  Branch40-48/RConn3 -- Bus48/RConn3 -- Branch48-48/LConn3 -- Branch47-48/RConn3
  Branch45-51/RConn1 -- Bus51/RConn1 -- Branch51-51/LConn1 -- Branch50-51/RConn1
  Branch45-51/RConn2 -- Bus51/RConn2 -- Branch51-51/LConn2 -- Branch50-51/RConn2
  Branch45-51/RConn3 -- Bus51/RConn3 -- Branch51-51/LConn3 -- Branch50-51/RConn3
  Branch47-48/LConn1 -- Bus47/RConn1 -- Branch47-47/LConn1 -- Branch47-53/LConn1
  Branch47-48/LConn2 -- Bus47/RConn2 -- Branch47-47/LConn2 -- Branch47-53/LConn2
  Branch47-48/LConn3 -- Bus47/RConn3 -- Branch47-47/LConn3 -- Branch47-53/LConn3
  Branch52-55/RConn1 -- Bus55/RConn1 -- Branch55-55/LConn1 -- Branch55-56/LConn1 -- Branch54-55/RConn1
  Branch52-55/RConn2 -- Bus55/RConn2 -- Branch55-55/LConn2 -- Branch55-56/LConn2 -- Branch54-55/RConn2
  Branch52-55/RConn3 -- Bus55/RConn3 -- Branch55-55/LConn3 -- Branch55-56/LConn3 -- Branch54-55/RConn3
  Branch55-56/RConn1 -- Bus56/RConn1 -- Branch56-56/LConn1 -- Branch56-66/LConn1 -- Branch56-57/LConn1
  Branch55-56/RConn2 -- Bus56/RConn2 -- Branch56-56/LConn2 -- Branch56-66/LConn2 -- Branch56-57/LConn2
  Branch55-56/RConn3 -- Bus56/RConn3 -- Branch56-56/LConn3 -- Branch56-66/LConn3 -- Branch56-57/LConn3
  Branch56-57/RConn1 -- Bus57/RConn1 -- Branch57-57/LConn1 -- Branch57-60/LConn1 -- Branch57-58/LConn1
  Branch56-57/RConn2 -- Bus57/RConn2 -- Branch57-57/LConn2 -- Branch57-60/LConn2 -- Branch57-58/LConn2
  Branch56-57/RConn3 -- Bus57/RConn3 -- Branch57-57/LConn3 -- Branch57-60/LConn3 -- Branch57-58/LConn3
  Branch56-66/RConn1 -- Bus66/RConn1 -- Branch66-66/LConn1 -- Branch66-67/LConn1 -- Branch65-66/RConn1
  Branch56-66/RConn2 -- Bus66/RConn2 -- Branch66-66/LConn2 -- Branch66-67/LConn2 -- Branch65-66/RConn2
  Branch56-66/RConn3 -- Bus66/RConn3 -- Branch66-66/LConn3 -- Branch66-67/LConn3 -- Branch65-66/RConn3
  Branch57-60/RConn1 -- Bus60/RConn1 -- Branch60-60/LConn1 -- Branch60-61/LConn1 -- Branch59-60/RConn1
  Branch57-60/RConn2 -- Bus60/RConn2 -- Branch60-60/LConn2 -- Branch60-61/LConn2 -- Branch59-60/RConn2
  Branch57-60/RConn3 -- Bus60/RConn3 -- Branch60-60/LConn3 -- Branch60-61/LConn3 -- Branch59-60/RConn3
  Branch58-59/RConn1 -- Bus59/RConn1 -- Branch59-59/LConn1 -- Branch59-60/LConn1
  Branch58-59/RConn2 -- Bus59/RConn2 -- Branch59-59/LConn2 -- Branch59-60/LConn2
  Branch58-59/RConn3 -- Bus59/RConn3 -- Branch59-59/LConn3 -- Branch59-60/LConn3
  Branch58-63/RConn1 -- Bus63/RConn1 -- Branch63-63/LConn1 -- Transformer63-64/LConn1 -- Branch62-63/RConn1
  Branch58-63/RConn2 -- Bus63/RConn2 -- Branch63-63/LConn2 -- Transformer63-64/LConn2 -- Branch62-63/RConn2
  Branch58-63/RConn3 -- Bus63/RConn3 -- Branch63-63/LConn3 -- Transformer63-64/LConn3 -- Branch62-63/RConn3
  Branch62-65/RConn1 -- Bus65/RConn1 -- Branch65-65/LConn1 -- Branch65-66/LConn1 -- Branch64-65/RConn1
  Branch62-65/RConn2 -- Bus65/RConn2 -- Branch65-65/LConn2 -- Branch65-66/LConn2 -- Branch64-65/RConn2
  Branch62-65/RConn3 -- Bus65/RConn3 -- Branch65-65/LConn3 -- Branch65-66/LConn3 -- Branch64-65/RConn3
  Branch63-64/RConn1 -- Bus64/RConn1 -- Branch64-64/LConn1 -- Transformer64-65/LConn1
  Branch63-64/RConn2 -- Bus64/RConn2 -- Branch64-64/LConn2 -- Transformer64-65/LConn2
  Branch63-64/RConn3 -- Bus64/RConn3 -- Branch64-64/LConn3 -- Transformer64-65/LConn3
  Transformer63-64/RConn1 -- Branch63-64/LConn1
  Transformer63-64/RConn2 -- Branch63-64/LConn2
  Transformer63-64/RConn3 -- Branch63-64/LConn3
  Transformer64-65/RConn1 -- Branch64-65/LConn1
  Transformer64-65/RConn2 -- Branch64-65/LConn2
  Transformer64-65/RConn3 -- Branch64-65/LConn3
  Branch66-67/RConn1 -- Bus67/RConn1 -- Branch67-67/LConn1 -- Branch67-68/LConn1
  Branch66-67/RConn2 -- Bus67/RConn2 -- Branch67-67/LConn2 -- Branch67-68/LConn2
  Branch66-67/RConn3 -- Bus67/RConn3 -- Branch67-67/LConn3 -- Branch67-68/LConn3
  SM_8th_GOV1/LConn1 -- Bus1/LConn1
  SM_8th_GOV1/LConn2 -- Bus1/LConn2
  SM_8th_GOV1/LConn3 -- Bus1/LConn3
  SM_8th_AVRPSSGOV2/LConn1 -- Bus2/LConn1
  SM_8th_AVRPSSGOV2/LConn2 -- Bus2/LConn2
  SM_8th_AVRPSSGOV2/LConn3 -- Bus2/LConn3
  SM_8th_AVRPSSGOV3/LConn1 -- Bus3/LConn1
  SM_8th_AVRPSSGOV3/LConn2 -- Bus3/LConn2
  SM_8th_AVRPSSGOV3/LConn3 -- Bus3/LConn3
  SM_8th_AVRPSSGOV4/LConn1 -- Bus4/LConn1
  SM_8th_AVRPSSGOV4/LConn2 -- Bus4/LConn2
  SM_8th_AVRPSSGOV4/LConn3 -- Bus4/LConn3
  SM_8th_AVRPSSGOV5/LConn1 -- Bus5/LConn1
  SM_8th_AVRPSSGOV5/LConn2 -- Bus5/LConn2
  SM_8th_AVRPSSGOV5/LConn3 -- Bus5/LConn3
  SM_8th_AVRPSSGOV6/LConn1 -- Bus6/LConn1
  SM_8th_AVRPSSGOV6/LConn2 -- Bus6/LConn2
  SM_8th_AVRPSSGOV6/LConn3 -- Bus6/LConn3
  SM_8th_AVRPSSGOV7/LConn1 -- Bus7/LConn1
  SM_8th_AVRPSSGOV7/LConn2 -- Bus7/LConn2
  SM_8th_AVRPSSGOV7/LConn3 -- Bus7/LConn3
  SM_8th_AVRPSSGOV8/LConn1 -- Bus8/LConn1
  SM_8th_AVRPSSGOV8/LConn2 -- Bus8/LConn2
  SM_8th_AVRPSSGOV8/LConn3 -- Bus8/LConn3
  SM_8th_AVRPSSGOV9/LConn1 -- Bus9/LConn1
  SM_8th_AVRPSSGOV9/LConn2 -- Bus9/LConn2
  SM_8th_AVRPSSGOV9/LConn3 -- Bus9/LConn3
  SM_8th_AVRPSSGOV10/LConn1 -- Bus10/LConn1
  SM_8th_AVRPSSGOV10/LConn2 -- Bus10/LConn2
  SM_8th_AVRPSSGOV10/LConn3 -- Bus10/LConn3
  SM_8th_AVRPSSGOV11/LConn1 -- Bus11/LConn1
  SM_8th_AVRPSSGOV11/LConn2 -- Bus11/LConn2
  SM_8th_AVRPSSGOV11/LConn3 -- Bus11/LConn3
  SM_8th_AVRPSSGOV12/LConn1 -- Bus12/LConn1
  SM_8th_AVRPSSGOV12/LConn2 -- Bus12/LConn2
  SM_8th_AVRPSSGOV12/LConn3 -- Bus12/LConn3
  SM_8th_GOV13/LConn1 -- Bus13/LConn1
  SM_8th_GOV13/LConn2 -- Bus13/LConn2
  SM_8th_GOV13/LConn3 -- Bus13/LConn3
  SM_8th_GOV14/LConn1 -- Bus14/LConn1
  SM_8th_GOV14/LConn2 -- Bus14/LConn2
  SM_8th_GOV14/LConn3 -- Bus14/LConn3
  SM_8th_GOV15/LConn1 -- Bus15/LConn1
  SM_8th_GOV15/LConn2 -- Bus15/LConn2
  SM_8th_GOV15/LConn3 -- Bus15/LConn3
  SM_8th_AVRPSSGOV16/LConn1 -- Bus16/LConn1
  SM_8th_AVRPSSGOV16/LConn2 -- Bus16/LConn2
  SM_8th_AVRPSSGOV16/LConn3 -- Bus16/LConn3
  VSI-PLL17/LConn1 -- Bus17/LConn1
  VSI-PLL17/LConn2 -- Bus17/LConn2
  VSI-PLL17/LConn3 -- Bus17/LConn3
  VSI-PLL26/LConn1 -- Bus26/LConn1
  VSI-PLL26/LConn2 -- Bus26/LConn2
  VSI-PLL26/LConn3 -- Bus26/LConn3
  VSI-PLL27/LConn1 -- Bus27/LConn1
  VSI-PLL27/LConn2 -- Bus27/LConn2
  VSI-PLL27/LConn3 -- Bus27/LConn3
  VSI-PLL28/LConn1 -- Bus28/LConn1
  VSI-PLL28/LConn2 -- Bus28/LConn2
  VSI-PLL28/LConn3 -- Bus28/LConn3
  VSI-PLL29/LConn1 -- Bus29/LConn1
  VSI-PLL29/LConn2 -- Bus29/LConn2
  VSI-PLL29/LConn3 -- Bus29/LConn3
  VSI-PLL35/LConn1 -- Bus35/LConn1
  VSI-PLL35/LConn2 -- Bus35/LConn2
  VSI-PLL35/LConn3 -- Bus35/LConn3
  VSI-PLL39/LConn1 -- Bus39/LConn1
  VSI-PLL39/LConn2 -- Bus39/LConn2
  VSI-PLL39/LConn3 -- Bus39/LConn3
  VSI-PLL43/LConn1 -- Bus43/LConn1
  VSI-PLL43/LConn2 -- Bus43/LConn2
  VSI-PLL43/LConn3 -- Bus43/LConn3
  VSI-PLL44/LConn1 -- Bus44/LConn1
  VSI-PLL44/LConn2 -- Bus44/LConn2
  VSI-PLL44/LConn3 -- Bus44/LConn3
  VSI-PLL45/LConn1 -- Bus45/LConn1
  VSI-PLL45/LConn2 -- Bus45/LConn2
  VSI-PLL45/LConn3 -- Bus45/LConn3
  VSI-PLL50/LConn1 -- Bus50/LConn1
  VSI-PLL50/LConn2 -- Bus50/LConn2
  VSI-PLL50/LConn3 -- Bus50/LConn3
  VSI-PLL51/LConn1 -- Bus51/LConn1
  VSI-PLL51/LConn2 -- Bus51/LConn2
  VSI-PLL51/LConn3 -- Bus51/LConn3
  VSI-PLL58/LConn1 -- Bus58/LConn1
  VSI-PLL58/LConn2 -- Bus58/LConn2
  VSI-PLL58/LConn3 -- Bus58/LConn3
  VSI-PLL59/LConn1 -- Bus59/LConn1
  VSI-PLL59/LConn2 -- Bus59/LConn2
  VSI-PLL59/LConn3 -- Bus59/LConn3
  Branch26-1/RConn3 -- Branch26-1/RConn1 -- B-GND2/LConn1 -- Branch26-1/RConn2
  Branch26-1/LConn2 -- Three-Phase Breaker/RConn2
  Branch26-1/LConn3 -- Three-Phase Breaker/RConn3
  Branch26-1/LConn1 -- Three-Phase Breaker/RConn1
  Branch26-2/RConn2 -- Branch26-2/RConn1 -- B-GND4/LConn1 -- Branch26-2/RConn3
  Branch26-2/LConn1 -- Three-Phase Breaker1/RConn1
  Branch26-2/LConn3 -- Three-Phase Breaker1/RConn3
  Branch26-2/LConn2 -- Three-Phase Breaker1/RConn2
  Branch26-3/RConn2 -- Branch26-3/RConn1 -- B-GND6/LConn1 -- Branch26-3/RConn3
  Branch26-3/LConn3 -- Three-Phase Breaker2/RConn3
  Branch26-3/LConn1 -- Three-Phase Breaker2/RConn1
  Branch26-3/LConn2 -- Three-Phase Breaker2/RConn2
